simulink model "ABB_1010"  (R2024a)
settings: Solver=VariableStepAuto  StartTime=0.0  StopTime=200  RelTol=1e-3
model workspace: external: MATLAB File C:\Users\lucas\OneDrive\Documents\MATLAB\projeto final\ABB_1010_DataFile.m (data not in the file)
values from neighbouring files (symbols this model uses):
  g = 9.81    [inicializacaoAntropomorfico.m]
  I1 = [ 0.00243841  0.00000307  0.00007261    [inicializacaoAntropomorfico.m]
  I2 = [ 0.01633569  0.00000387 -0.00034405    [inicializacaoAntropomorfico.m]
  I3 = [ 0.00244760 -0.00000208  0.00000538    [inicializacaoAntropomorfico.m]
  I4 = [ 0.00245792 -0.00000008  0.00003121    [inicializacaoAntropomorfico.m]
  I5 = [ 0.00062165 -0.00000206 -0.00000303    [inicializacaoAntropomorfico.m]
  I6 = [ 0.00000357  0.00000000  0.00000000    [inicializacaoAntropomorfico.m]
  I7 = [(m7*L7^2)/12 0.00000000  0.00000000    [inicializacaoAntropomorfico.m]
  L = [L1, L2, L3, L4, L5, L6, L7]    [inicializacaoAntropomorfico.m]
  Lcm1 = [-0.00258308  0.00024508 -0.01434968]    [inicializacaoAntropomorfico.m]
  Lcm2 = [-0.02078894  0.00020016 -0.10516734]    [inicializacaoAntropomorfico.m]
  Lcm3 = [ 0.00021912  0.00015355 -0.06228290]    [inicializacaoAntropomorfico.m]
  Lcm4 = [-0.00172658 -0.00124140 -0.07369196]    [inicializacaoAntropomorfico.m]
  Lcm5 = [-0.00014110  0.00085992 -0.03825278]    [inicializacaoAntropomorfico.m]
  Lcm6 = [ 0.00002478  0.00000000 -0.00042157]    [inicializacaoAntropomorfico.m]
  Lcm7 = [ 0           0          -0.05000000]    [inicializacaoAntropomorfico.m]
  m = [m1, m2, m3, m4, m5, m6, m7]    [inicializacaoAntropomorfico.m]
  Pf = [  0.05    [inicializacaoAntropomorfico.m]
  Pi = [  0.2    [inicializacaoAntropomorfico.m]
  Raio = [0]    [inicializacaoAntropomorfico.m]
  Sentido = [0]    [inicializacaoAntropomorfico.m]
  Tipo = [1]    [inicializacaoAntropomorfico.m]
undefined symbols (not defined in the file or in its folder): smiData, X, Y, Z
libraries: sm_lib x35, nesl_utility x7
(part 6 of 16)

== matlab function ABB_1010/Dinamica/MATLAB Function1 ==
  data: H output; Q input; I1 parameter; I2 parameter; L parameter; Lcm1 parameter; Lcm2 parameter; Lcm3 parameter; Lcm4 parameter; Lcm5 parameter; Lcm6 parameter; I6 parameter; I5 parameter; I4 parameter; I3 parameter; dQ input; m parameter
function H = func_H(Q, I1, I2, L, Lcm1, Lcm2, Lcm3, Lcm4, Lcm5, Lcm6, I6, I5, I4, I3, dQ, m)
%func_H
%    OUT1 = func_H(Ixx2,Ixx3,Ixx4,Ixx5,Ixx6,Ixy2,Ixy3,Ixy4,Ixy5,Ixy6,Ixz2,Ixz3,Ixz4,Ixz5,Ixz6,Iyx2,Iyx3,Iyx4,Iyx5,Iyx6,Iyy4,Iyy5,Iyy6,Iyz2,Iyz3,Iyz4,Iyz5,Iyz6,Izx2,Izx3,Izx4,Izx5,Izx6,Izy2,Izy3,Izy4,Izy5,Izy6,Izz2,Izz3,Izz4,Izz5,Izz6,Lx2,Lx3,Lxcm2,Lxcm3,Lxcm4,Lxcm5,Lxcm6,Lycm2,Lycm3,Lycm4,Lycm5,Lycm6,Lz4,Lz5,Lzcm2,Lzcm3,Lzcm4,Lzcm5,Lzcm6,Q1,Q2,Q3,Q4,Q5,Q6,dQ1,dQ2,dQ3,dQ4,dQ5,dQ6,M2,M3,M4,M5,M6)

%    This function was generated by the Symbolic Math Toolbox version 24.1.
%    30-Apr-2025 06:22:27

m1  = m(1);
m2  = m(2);
m3  = m(3);
m4  = m(4);
m5  = m(5);
m6  = m(6);

Q1  = Q(1);
Q2  = Q(2);
Q3  = Q(3);
Q4  = Q(4);
Q5  = Q(5);
Q6  = Q(6);

dQ1 = dQ(1);
dQ2 = dQ(2);
dQ3 = dQ(3);
dQ4 = dQ(4);
dQ5 = dQ(5);
dQ6 = dQ(6);

Lz1 = L(1);
Lx2 = L(2);
Lx3 = L(3);
Lz4 = L(4);
Lz5 = L(5);
Lz6 = L(6);

Lxcm1 = Lcm1(1);
Lycm1 = Lcm1(2);
Lzcm1 = Lcm1(3);

Lxcm2 = Lcm2(1);
Lycm2 = Lcm2(2);
Lzcm2 = Lcm2(3);

Lxcm3 = Lcm3(1);
Lycm3 = Lcm3(2);
Lzcm3 = Lcm3(3);

Lxcm4 = Lcm4(1);
Lycm4 = Lcm4(2);
Lzcm4 = Lcm4(3);

Lxcm5 = Lcm5(1);
Lycm5 = Lcm5(2);
Lzcm5 = Lcm5(3);

Lxcm6 = Lcm6(1);
Lycm6 = Lcm6(2);
Lzcm6 = Lcm6(3);

Ixx1 = I1(1,1);
Ixy1 = I1(1,2);
Ixz1 = I1(1,3);
Iyx1 = I1(2,1);
Iyy1 = I1(2,2);
Iyz1 = I1(2,3);
Izx1 = I1(3,1);
Izy1 = I1(3,2);
Izz1 = I1(3,3);

Ixx2 = I2(1,1);
Ixy2 = I2(1,2);
Ixz2 = I2(1,3);
Iyx2 = I2(2,1);
Iyy2 = I2(2,2);
Iyz2 = I2(2,3);
Izx2 = I2(3,1);
Izy2 = I2(3,2);
Izz2 = I2(3,3);

Ixx3 = I3(1,1);
Ixy3 = I3(1,2);
Ixz3 = I3(1,3);
Iyx3 = I3(2,1);
Iyy3 = I3(2,2);
Iyz3 = I3(2,3);
Izx3 = I3(3,1);
Izy3 = I3(3,2);
Izz3 = I3(3,3);

Ixx4 = I4(1,1);
Ixy4 = I4(1,2);
Ixz4 = I4(1,3);
Iyx4 = I4(2,1);
Iyy4 = I4(2,2);
Iyz4 = I4(2,3);
Izx4 = I4(3,1);
Izy4 = I4(3,2);
Izz4 = I4(3,3);

Ixx5 = I5(1,1);
Ixy5 = I5(1,2);
Ixz5 = I5(1,3);
Iyx5 = I5(2,1);
Iyy5 = I5(2,2);
Iyz5 = I5(2,3);
Izx5 = I5(3,1);
Izy5 = I5(3,2);
Izz5 = I5(3,3);

Ixx6 = I6(1,1);
Ixy6 = I6(1,2);
Ixz6 = I6(1,3);
Iyx6 = I6(2,1);
Iyy6 = I6(2,2);
Iyz6 = I6(2,3);
Izx6 = I6(3,1);
Izy6 = I6(3,2);
Izz6 = I6(3,3);


t2 = cos(Q1);
t3 = cos(Q2);
t4 = cos(Q3);
t5 = cos(Q4);
t6 = cos(Q5);
t7 = cos(Q6);
t8 = sin(Q1);
t9 = sin(Q2);
t10 = sin(Q3);
t11 = sin(Q4);
t12 = sin(Q5);
t13 = sin(Q6);
t14 = Q2+Q3;
t15 = Lxcm4.^2;
t16 = Lxcm5.^2;
t17 = Lxcm6.^2;
t18 = Lycm4.^2;
t19 = Lycm5.^2;
t20 = Lycm6.^2;
t21 = Lz5.^2;
t22 = Lzcm5.^2;
t23 = Lzcm6.^2;
t24 = Q4.*2.0;
t25 = Q5.*2.0;
t26 = Q6.*2.0;
t27 = dQ1.^2;
t28 = dQ2.^2;
t29 = dQ3.^2;
t30 = dQ4.^2;
t31 = dQ5.^2;
t32 = dQ6.^2;
t33 = cos(t24);
t34 = cos(t25);
t35 = cos(t26);
t36 = t5.^2;
t37 = t6.^2;
t38 = t7.^2;
t39 = sin(t26);
t40 = t11.^2;
t41 = t12.^2;
t42 = t13.^2;
t43 = Lycm3.*t2;
t44 = Lzcm2.*t3;
t45 = cos(t14);
t46 = Lx2.*t9;
t47 = Lxcm2.*t9;
t48 = Lycm3.*t8;
t49 = sin(t14);
t50 = t2.*t5;
t51 = Lz4.*m5.*t4;
t52 = Lz4.*m6.*t4;
t53 = Lzcm3.*m3.*t4;
t54 = Lzcm4.*m4.*t4;
t55 = t2.*t11;
t56 = t5.*t8;
t57 = Lx3.*m4.*t10;
t58 = Lx3.*m5.*t10;
t59 = Lx3.*m6.*t10;
t60 = Lxcm3.*m3.*t10;
t61 = t8.*t11;
t72 = Lx2.*t2.*t3;
t75 = Lx3.*Lycm4.*m4.*t5;
t76 = Lx3.*Lycm5.*m5.*t5;
t77 = Lx3.*Lz5.*m6.*t6;
t78 = Lx3.*Lzcm5.*m5.*t6;
t79 = Lxcm5.*Lz4.*m5.*t6;
t80 = Lx3.*Lzcm6.*m6.*t6;
t81 = Lxcm4.*Lzcm4.*m4.*t5;
t82 = Lxcm5.*Lzcm5.*m5.*t5;
t92 = Ixx4.*t5.*t11;
t93 = Ixx6.*t5.*t11;
t94 = Ixx5.*t6.*t12;
t95 = Iyy4.*t5.*t11;
t96 = Iyy5.*t5.*t11;
t97 = Iyy6.*t6.*t12;
t98 = Izz5.*t5.*t11;
t99 = Izz6.*t5.*t11;
t100 = Izz5.*t6.*t12;
t101 = Izz6.*t6.*t12;
t102 = Lx2.*t3.*t8;
t103 = Lx3.*t3.*t10;
t104 = Lx3.*t4.*t9;
t108 = Lx3.*Lxcm4.*m4.*t11;
t109 = Lx3.*Lxcm5.*m5.*t12;
t110 = Lycm5.*Lz4.*m5.*t11;
t111 = Lycm4.*Lzcm4.*m4.*t11;
t112 = Lz4.*Lz5.*m6.*t12;
t113 = Lz4.*Lzcm5.*m5.*t12;
t114 = Lz4.*Lzcm6.*m6.*t12;
t119 = (Ixz4.*t5)./2.0;
t120 = (Ixz5.*t5)./2.0;
t121 = (Izx4.*t5)./2.0;
t122 = (Izx5.*t5)./2.0;
t123 = (Iyz4.*t11)./2.0;
t124 = (Izy4.*t11)./2.0;
t126 = t2.*t3.*t4;
t127 = Lz5.*m6.*t4.*t6;
t128 = Lzcm5.*m5.*t4.*t6;
t129 = Lzcm6.*m6.*t4.*t6;
t132 = t2.*t3.*t10;
t133 = t2.*t4.*t9;
t134 = t3.*t4.*t8;
t135 = Lxcm4.*m4.*t5.*t10;
t136 = Lxcm5.*m5.*t4.*t12;
t138 = t2.*t9.*t10;
t139 = t3.*t8.*t10;
t140 = t4.*t8.*t9;
t141 = Lycm4.*m4.*t10.*t11;
t142 = Lycm5.*m5.*t10.*t11;
t143 = t8.*t9.*t10;
t193 = Lx3.*Lycm6.*m6.*t5.*t7;
t198 = Lxcm6.*Lz4.*m6.*t6.*t7;
t199 = Lxcm6.*Lz5.*m6.*t5.*t7;
t200 = Lxcm6.*Lzcm6.*m6.*t5.*t7;
t230 = Lxcm4.*t3.*t5.*t10;
t231 = Lxcm4.*t4.*t5.*t9;
t236 = Lx3.*Lxcm5.*m5.*t6.*t11;
t237 = Lx3.*Lxcm6.*m6.*t5.*t13;
t238 = Lx3.*Lxcm6.*m6.*t7.*t11;
t239 = Lx3.*Lxcm6.*m6.*t7.*t12;
t240 = Lycm6.*Lz4.*m6.*t7.*t11;
t241 = Lycm6.*Lz4.*m6.*t6.*t13;
t242 = Lycm6.*Lz4.*m6.*t7.*t12;
t243 = Lycm6.*Lz5.*m6.*t5.*t13;
t244 = Lycm6.*Lz5.*m6.*t7.*t12;
t245 = Lycm5.*Lzcm5.*m5.*t6.*t11;
t246 = Lycm6.*Lzcm6.*m6.*t5.*t13;
t247 = Lycm6.*Lzcm6.*m6.*t7.*t12;
t266 = Lycm4.*t3.*t10.*t11;
t267 = Lycm4.*t4.*t9.*t11;
t268 = Lycm5.*t3.*t10.*t11;
t269 = Lycm5.*t4.*t9.*t11;
t273 = Lx3.*Lycm6.*m6.*t11.*t13;
t274 = Lx3.*Lycm6.*m6.*t12.*t13;
t275 = Lxcm5.*Lycm5.*m5.*t11.*t12;
t276 = Lxcm6.*Lycm6.*m6.*t11.*t12;
t277 = Lx3.*Lz5.*m6.*t11.*t12;
t278 = Lx3.*Lzcm5.*m5.*t11.*t12;
t279 = Lx3.*Lzcm6.*m6.*t11.*t12;
t280 = Lxcm6.*Lz4.*m6.*t11.*t13;
t281 = Lxcm6.*Lz4.*m6.*t12.*t13;
t282 = Lxcm6.*Lz5.*m6.*t12.*t13;
t283 = Lxcm6.*Lzcm6.*m6.*t12.*t13;
t288 = (Ixz6.*t5.*t7)./2.0;
t289 = (Izx6.*t5.*t7)./2.0;
t290 = (Iyz5.*t6.*t11)./2.0;
t291 = (Iyz6.*t5.*t13)./2.0;
t292 = (Iyz6.*t7.*t12)./2.0;
t293 = (Izy5.*t6.*t11)./2.0;
t294 = (Izy6.*t5.*t13)./2.0;
t295 = (Izy6.*t7.*t12)./2.0;
t297 = (Ixy5.*t11.*t12)./2.0;
t298 = (Ixy6.*t11.*t12)./2.0;
t299 = (Ixz6.*t12.*t13)./2.0;
t300 = (Iyx5.*t11.*t12)./2.0;
t301 = (Iyx6.*t11.*t12)./2.0;
t302 = (Izx6.*t12.*t13)./2.0;
t308 = Lxcm5.*m5.*t5.*t6.*t10;
t309 = Lxcm6.*m6.*t4.*t7.*t12;
t316 = Lycm6.*m6.*t7.*t10.*t11;
t317 = Lycm6.*m6.*t4.*t12.*t13;
t318 = Lz5.*m6.*t5.*t10.*t12;
t319 = Lzcm5.*m5.*t5.*t10.*t12;
t320 = Lzcm6.*m6.*t5.*t10.*t12;
t323 = Lxcm6.*m6.*t10.*t11.*t13;
t334 = Lz5.*Lzcm6.*m6.*t5.*t11.*2.0;
t335 = Lz5.*Lzcm6.*m6.*t6.*t12.*2.0;
t336 = m4.*t5.*t11.*t15;
t337 = m5.*t6.*t12.*t16;
t338 = m6.*t5.*t11.*t17;
t339 = m4.*t5.*t11.*t18;
t340 = m5.*t5.*t11.*t19;
t341 = m6.*t6.*t12.*t20;
t342 = m6.*t5.*t11.*t21;
t343 = m6.*t6.*t12.*t21;
t344 = m5.*t5.*t11.*t22;
t345 = m5.*t6.*t12.*t22;
t346 = m6.*t5.*t11.*t23;
t347 = m6.*t6.*t12.*t23;
t417 = Lxcm5.*t3.*t5.*t6.*t10;
t418 = Lxcm5.*t4.*t5.*t6.*t9;
t428 = Lycm6.*Lz5.*m6.*t6.*t7.*t11;
t431 = Lycm6.*Lzcm6.*m6.*t6.*t7.*t11;
t456 = Ixy6.*t5.*t7.*t11.*t13;
t457 = Ixy6.*t6.*t7.*t12.*t13;
t458 = Ixz5.*t5.*t6.*t11.*t12;
t459 = Iyx6.*t5.*t7.*t11.*t13;
t460 = Iyx6.*t6.*t7.*t12.*t13;
t461 = Izx5.*t5.*t6.*t11.*t12;
t467 = Lzcm5.*t3.*t5.*t10.*t12;
t468 = Lzcm5.*t4.*t5.*t9.*t12;
t478 = Lxcm6.*Lz5.*m6.*t6.*t11.*t13;
t480 = Lxcm6.*Lzcm6.*m6.*t6.*t11.*t13;
t489 = Ixx6.*t7.*t11.*t12.*t13;
t490 = Iyy6.*t7.*t11.*t12.*t13;
t538 = Lycm6.*m6.*t5.*t6.*t10.*t13;
t578 = (Iyz6.*t6.*t7.*t11)./2.0;
t581 = (Izy6.*t6.*t7.*t11)./2.0;
t586 = (Ixz6.*t6.*t11.*t13)./2.0;
t590 = (Izx6.*t6.*t11.*t13)./2.0;
t599 = Lxcm6.*m6.*t5.*t6.*t7.*t10;
t648 = Ixz6.*t5.*t6.*t7.*t11.*t12;
t650 = Izx6.*t5.*t6.*t7.*t11.*t12;
t667 = Iyz6.*t5.*t6.*t11.*t12.*t13;
t668 = Izy6.*t5.*t6.*t11.*t12.*t13;
t711 = Lz5.*Lzcm6.*m6.*t5.*t6.*t12.*-2.0;
t742 = Ixy5.*t5.*t11.*t12.*(-1.0./2.0);
t743 = Iyx5.*t5.*t11.*t12.*(-1.0./2.0);
t788 = Lxcm6.*Lycm6.*m6.*t5.*t7.*t11.*t13.*2.0;
t789 = Lxcm6.*Lycm6.*m6.*t6.*t7.*t12.*t13.*2.0;
t791 = m6.*t7.*t11.*t12.*t13.*t17;
t792 = m6.*t7.*t11.*t12.*t13.*t20;
t886 = Ixz6.*t5.*t7.*t11.*t12.*(-1.0./2.0);
t887 = Izx6.*t5.*t7.*t11.*t12.*(-1.0./2.0);
t928 = Lxcm6.*Lycm6.*m6.*t5.*t6.*t7.*t11.*t13.*4.0;
t968 = Lxcm6.*Lycm6.*m6.*t5.*t6.*t7.*t12.*t13.*-2.0;
t62 = Ixx3.*t45;
t63 = Ixz3.*t45;
t64 = Izx3.*t45;
t65 = Izx4.*t45;
t66 = Izy4.*t45;
t67 = Izz3.*t45;
t68 = Izz4.*t45;
t69 = Lz4.*t45;
t70 = Lzcm3.*t45;
t71 = Lzcm4.*t45;
t73 = Lycm4.*t50;
t74 = Lycm5.*t50;
t83 = Ixx3.*t49;
t84 = Ixz3.*t49;
t85 = Izx3.*t49;
t86 = Izx4.*t49;
t87 = Izy4.*t49;
t88 = Izz3.*t49;
t89 = Izz4.*t49;
t90 = Lx3.*t49;
t91 = Lxcm3.*t49;
t105 = Lxcm4.*t55;
t106 = Lycm4.*t56;
t107 = Lycm5.*t56;
t115 = Lxcm4.*t61;
t116 = -t46;
t117 = -t47;
t118 = -t48;
t125 = t6.*t45;
t130 = t12.*t45;
t131 = t6.*t49;
t137 = t12.*t49;
t144 = -t50;
t145 = -t57;
t146 = -t58;
t147 = -t59;
t148 = -t60;
t149 = -t61;
t154 = -t77;
t155 = -t78;
t156 = -t80;
t157 = -t81;
t163 = -t92;
t164 = -t98;
t165 = -t99;
t166 = -t100;
t167 = -t101;
t171 = -t119;
t172 = -t121;
t173 = Ixz5.*t5.*t37;
t174 = Izx5.*t5.*t37;
t175 = Lxcm4.*Lycm4.*m4.*t33;
t176 = Lxcm6.*Lycm6.*m6.*t35;
t177 = Lxcm5.*Lzcm5.*m5.*t34;
t178 = Ixx4.*t5.*t45;
t179 = Ixy4.*t5.*t45;
t180 = Ixz4.*t5.*t45;
t186 = Lx3.*t2.*t45;
t187 = Lxcm3.*t2.*t45;
t191 = Lx3.*t126;
t192 = Lycm6.*t7.*t50;
t196 = t5.*t79;
t201 = Ixx4.*t5.*t49;
t203 = Ixy4.*t5.*t49;
t205 = Ixz4.*t5.*t49;
t207 = Iyx4.*t11.*t45;
t208 = Iyx5.*t11.*t45;
t209 = Iyy4.*t11.*t45;
t210 = Iyy5.*t11.*t45;
t211 = Iyz4.*t11.*t45;
t212 = Iyz5.*t11.*t45;
t219 = Lx3.*t8.*t45;
t220 = Lxcm3.*t8.*t45;
t222 = Lz4.*t2.*t49;
t223 = Lzcm3.*t2.*t49;
t224 = Lzcm4.*t2.*t49;
t225 = t5.*t94;
t226 = t5.*t97;
t227 = t5.*t100;
t228 = t5.*t101;
t229 = Lx3.*t134;
t232 = Lxcm5.*t6.*t55;
t233 = Lxcm6.*t13.*t50;
t234 = Lycm6.*t7.*t56;
t235 = t5.*t109;
t248 = t5.*t112;
t249 = t5.*t113;
t250 = t5.*t114;
t254 = Iyx4.*t11.*t49;
t255 = Iyx5.*t11.*t49;
t256 = Iyy4.*t11.*t49;
t257 = Iyy5.*t11.*t49;
t258 = Iyz4.*t11.*t49;
t259 = Iyz5.*t11.*t49;
t260 = Lz4.*t8.*t49;
t261 = Lzcm3.*t8.*t49;
t262 = Lzcm4.*t8.*t49;
t263 = Lx3.*t138;
t264 = Lxcm5.*t6.*t61;
t265 = Lxcm6.*t13.*t56;
t270 = Lz5.*t12.*t55;
t271 = Lzcm5.*t12.*t55;
t272 = Lzcm6.*t12.*t55;
t284 = Lx3.*t143;
t286 = Lzcm5.*t12.*t61;
t305 = t7.*t11.*t45;
t306 = t5.*t7.*t49;
t311 = t11.*t13.*t45;
t312 = t5.*t13.*t49;
t313 = t7.*t11.*t49;
t321 = t11.*t13.*t49;
t324 = -t135;
t325 = -t136;
t326 = -t138;
t327 = -t143;
t328 = (Ixy4.*t33)./2.0;
t329 = (Ixy6.*t35)./2.0;
t330 = (Ixz5.*t34)./2.0;
t331 = (Iyx4.*t33)./2.0;
t332 = (Iyx6.*t35)./2.0;
t333 = (Izx5.*t34)./2.0;
t348 = -t288;
t349 = -t289;
t350 = -t291;
t351 = -t294;
t352 = Ixz6.*t5.*t7.*t37;
t353 = Izx6.*t5.*t7.*t37;
t354 = Lxcm5.*Lycm5.*m5.*t6.*t36;
t355 = Lxcm6.*Lycm6.*m6.*t6.*t36;
t356 = Lxcm6.*Lz5.*m6.*t7.*t37;
t357 = Lxcm6.*Lzcm6.*m6.*t7.*t37;
t358 = -t297;
t359 = -t300;
t360 = Ixx5.*t5.*t11.*t37;
t361 = t36.*t94;
t362 = t38.*t93;
t363 = Ixx6.*t6.*t12.*t38;
t364 = Ixx6.*t7.*t13.*t36;
t365 = Ixx6.*t7.*t13.*t37;
t366 = Iyy6.*t5.*t11.*t37;
t367 = Iyy6.*t5.*t11.*t38;
t368 = t36.*t97;
t369 = t38.*t97;
t370 = Iyy6.*t7.*t13.*t36;
t371 = Iyy6.*t7.*t13.*t37;
t372 = Iyz6.*t5.*t13.*t37;
t373 = Izy6.*t5.*t13.*t37;
t374 = t37.*t98;
t375 = t36.*t100;
t376 = t37.*t99;
t377 = t36.*t101;
t378 = Lxcm5.*Lycm5.*m5.*t6.*t40;
t379 = Lxcm6.*Lycm6.*m6.*t6.*t40;
t380 = Lxcm6.*Lz5.*m6.*t7.*t41;
t381 = Lxcm6.*Lzcm6.*m6.*t7.*t41;
t382 = Lycm6.*Lz5.*m6.*t13.*t37;
t383 = Lycm5.*Lzcm5.*m5.*t12.*t36;
t384 = Lycm6.*Lzcm6.*m6.*t13.*t37;
t385 = Ixy6.*t11.*t12.*t38;
t386 = Iyx6.*t11.*t12.*t38;
t387 = Lycm6.*Lz5.*m6.*t13.*t41;
t388 = Lycm5.*Lzcm5.*m5.*t12.*t40;
t389 = Lycm6.*Lzcm6.*m6.*t13.*t41;
t395 = Lxcm4.*t3.*t4.*t50;
t396 = t6.*t193;
t397 = t5.*t198;
t416 = Lxcm4.*t3.*t4.*t56;
t419 = Lxcm6.*t6.*t7.*t55;
t420 = Lycm4.*t3.*t4.*t55;
t421 = Lycm5.*t3.*t4.*t55;
t422 = Lx2.*t308;
t423 = Lx2.*t309;
t424 = t6.*t237;
t425 = t5.*t239;
t426 = t6.*t238;
t427 = t5.*t241;
t429 = t6.*t244;
t430 = t5.*t245;
t432 = t6.*t247;
t466 = Lycm6.*t6.*t13.*t55;
t469 = Lx2.*t316;
t470 = Lx2.*t317;
t471 = t5.*t274;
t472 = t6.*t273;
t473 = t5.*t275;
t474 = t5.*t276;
t475 = Lx2.*t318;
t476 = Lx2.*t319;
t477 = Lx2.*t320;
t479 = t6.*t282;
t481 = t6.*t283;
t491 = Lxcm4.*t9.*t10.*t56;
t492 = Lycm4.*t9.*t10.*t55;
t493 = Lycm5.*t9.*t10.*t55;
t494 = Lycm6.*t6.*t13.*t61;
t495 = Lx2.*t323;
t496 = Lycm4.*t9.*t10.*t61;
t497 = Lycm5.*t9.*t10.*t61;
t506 = -t199;
t507 = -t200;
t512 = -t238;
t513 = -t239;
t514 = -t241;
t515 = -t243;
t516 = -t246;
t526 = -t266;
t527 = -t267;
t528 = -t268;
t529 = -t269;
t530 = -t274;
t531 = -t275;
t541 = t37.*t82.*2.0;
t543 = -t308;
t544 = -t309;
t546 = -t318;
t547 = -t319;
t548 = -t320;
t551 = (Ixy5.*t6.*t36)./2.0;
t552 = (Ixy6.*t6.*t36)./2.0;
t553 = (Ixz6.*t7.*t37)./2.0;
t554 = (Iyx5.*t6.*t36)./2.0;
t555 = (Iyx6.*t6.*t36)./2.0;
t556 = (Izx6.*t7.*t37)./2.0;
t557 = (Ixy5.*t6.*t40)./2.0;
t558 = (Ixy6.*t6.*t40)./2.0;
t559 = (Ixz6.*t7.*t41)./2.0;
t560 = (Iyx5.*t6.*t40)./2.0;
t561 = (Iyx6.*t6.*t40)./2.0;
t562 = (Iyz5.*t12.*t36)./2.0;
t563 = (Iyz6.*t13.*t37)./2.0;
t564 = (Izx6.*t7.*t41)./2.0;
t565 = (Izy5.*t12.*t36)./2.0;
t566 = (Izy6.*t13.*t37)./2.0;
t567 = (Iyz5.*t12.*t40)./2.0;
t568 = (Iyz6.*t13.*t41)./2.0;
t569 = (Izy5.*t12.*t40)./2.0;
t570 = (Izy6.*t13.*t41)./2.0;
t572 = t5.*t337;
t573 = t5.*t341;
t574 = t5.*t343;
t575 = t5.*t345;
t576 = t5.*t347;
t577 = t5.*t290;
t579 = t6.*t292;
t580 = t5.*t293;
t582 = t6.*t295;
t585 = t5.*t298;
t587 = t6.*t299;
t589 = t5.*t301;
t591 = t6.*t302;
t592 = -t337;
t593 = -t338;
t594 = -t339;
t595 = -t340;
t596 = -t341;
t600 = t36.*t282;
t601 = t36.*t283;
t602 = t40.*t244;
t603 = t40.*t247;
t604 = t40.*t282;
t605 = t40.*t283;
t613 = Lxcm5.*t3.*t4.*t6.*t50;
t633 = Lxcm5.*t3.*t4.*t6.*t56;
t634 = Lycm6.*t3.*t4.*t7.*t55;
t635 = Lz5.*t3.*t4.*t12.*t50;
t636 = Lzcm5.*t3.*t4.*t12.*t50;
t637 = Lzcm6.*t3.*t4.*t12.*t50;
t640 = Lx2.*t599;
t641 = t5.*t428;
t642 = t5.*t431;
t647 = t5.*t457;
t649 = t5.*t460;
t652 = Lxcm6.*t3.*t4.*t13.*t55;
t653 = Lxcm6.*t7.*t12.*t132;
t654 = Lxcm6.*t7.*t12.*t133;
t656 = Lz5.*t3.*t4.*t12.*t56;
t657 = Lzcm5.*t3.*t4.*t12.*t56;
t658 = Lzcm6.*t3.*t4.*t12.*t56;
t659 = Lx2.*t538;
t660 = t5.*t478;
t661 = t11.*t12.*t199;
t662 = t5.*t480;
t663 = t11.*t12.*t200;
t665 = t7.*t12.*t13.*t93;
H = ft_1({Ixx2,Ixx4,Ixx5,Ixx6,Ixy2,Ixy3,Ixy4,Ixy5,Ixy6,Ixz2,Ixz4,Ixz5,Ixz6,Iyx2,Iyx3,Iyx4,Iyx5,Iyx6,Iyy4,Iyy5,Iyy6,Iyz2,Iyz3,Iyz4,Iyz5,Iyz6,Izx2,Izx4,Izx5,Izx6,Izy2,Izy3,Izy4,Izy5,Izy6,Izz2,Izz5,Izz6,Lx2,Lx3,Lxcm2,Lxcm3,Lxcm4,Lxcm5,Lxcm6,Lycm2,Lycm3,Lycm4,Lycm5,Lycm6,Lz4,Lz5,Lzcm2,Lzcm3,Lzcm4,Lzcm5,Lzcm6,m2,m3,m4,m5,m6,t10,t100,t101,t102,t103,t104,t105,t106,t107,t108,t109,t11,t110,t111,t112,t113,t114,t115,t116,t117,t118,t12,t120,t122,t123,t124,t125,t126,t127,t128,t129,t13,t130,t131,t132,t133,t134,t136,t137,t139,t140,t141,t142,t144,t145,t146,t147,t148,t149,t154,t155,t156,t157,t16,t163,t164,t165,t166,t167,t17,t171,t172,t173,t174,t175,t176,t177,t178,t179,t180,t186,t187,t191,t192,t193,t196,t198,t199,t2,t20,t200,t201,t203,t205,t207,t208,t209,t210,t211,t212,t219,t220,t222,t223,t224,t225,t226,t227,t228,t229,t230,t231,t232,t233,t234,t235,t236,t237,t239,t240,t241,t242,t243,t244,t245,t246,t247,t248,t249,t250,t254,t255,t256,t257,t258,t259,t260,t261,t262,t263,t264,t265,t27,t270,t271,t272,t273,t274,t276,t277,t278,t279,t28,t280,t281,t282,t283,t284,t286,t288,t289,t29,t290,t291,t292,t293,t294,t295,t298,t299,t3,t30,t301,t302,t305,t306,t31,t311,t312,t313,t316,t317,t32,t321,t323,t324,t325,t326,t327,t328,t329,t330,t331,t332,t333,t334,t335,t336,t337,t338,t339,t340,t341,t342,t343,t344,t345,t346,t347,t348,t349,t350,t351,t352,t353,t354,t355,t356,t357,t358,t359,t36,t360,t361,t362,t363,t364,t365,t366,t367,t368,t369,t37,t370,t371,t372,t373,t374,t375,t376,t377,t378,t379,t38,t380,t381,t382,t383,t384,t385,t386,t387,t388,t389,t39,t395,t396,t397,t4,t40,t41,t416,t417,t418,t419,t42,t420,t421,t422,t423,t424,t425,t426,t427,t428,t429,t43,t430,t431,t432,t44,t45,t456,t457,t458,t459,t46,t460,t461,t466,t467,t468,t469,t470,t471,t472,t473,t474,t475,t476,t477,t478,t479,t480,t481,t489,t49,t490,t491,t492,t493,t494,t495,t496,t497,t5,t50,t506,t507,t51,t512,t513,t514,t515,t516,t52,t526,t527,t528,t529,t53,t530,t531,t538,t54,t541,t543,t544,t546,t547,t548,t55,t551,t552,t553,t554,t555,t556,t557,t558,t559,t56,t560,t561,t562,t563,t564,t565,t566,t567,t568,t569,t57,t570,t572,t573,t574,t575,t576,t577,t578,t579,t58,t580,t581,t582,t585,t586,t587,t589,t59,t590,t591,t592,t593,t594,t595,t596,t599,t6,t600,t601,t602,t603,t604,t605,t61,t613,t62,t63,t633,t634,t635,t636,t637,t64,t640,t641,t642,t647,t648,t649,t65,t650,t652,t653,t654,t656,t657,t658,t659,t66,t660,t661,t662,t663,t665,t667,t668,t67,t68,t69,t7,t70,t71,t711,t72,t73,t74,t742,t743,t75,t76,t788,t789,t79,t791,t792,t8,t82,t83,t84,t85,t86,t87,t88,t886,t887,t89,t9,t90,t91,t92,t928,t93,t94,t95,t96,t968,t97,t98,t99});
end
function out1 = ft_1(ct)
[Ixx2,Ixx4,Ixx5,Ixx6,Ixy2,Ixy3,Ixy4,Ixy5,Ixy6,Ixz2,Ixz4,Ixz5,Ixz6,Iyx2,Iyx3,Iyx4,Iyx5,Iyx6,Iyy4,Iyy5,Iyy6,Iyz2,Iyz3,Iyz4,Iyz5,Iyz6,Izx2,Izx4,Izx5,Izx6,Izy2,Izy3,Izy4,Izy5,Izy6,Izz2,Izz5,Izz6,Lx2,Lx3,Lxcm2,Lxcm3,Lxcm4,Lxcm5,Lxcm6,Lycm2,Lycm3,Lycm4,Lycm5,Lycm6,Lz4,Lz5,Lzcm2,Lzcm3,Lzcm4,Lzcm5,Lzcm6,m2,m3,m4,m5,m6,t10,t100,t101,t102,t103,t104,t105,t106,t107,t108,t109,t11,t110,t111,t112,t113,t114,t115,t116,t117,t118,t12,t120,t122,t123,t124,t125,t126,t127,t128,t129,t13,t130,t131,t132,t133,t134,t136,t137,t139,t140,t141,t142,t144,t145,t146,t147,t148,t149,t154,t155,t156,t157,t16,t163,t164,t165,t166,t167,t17,t171,t172,t173,t174,t175,t176,t177,t178,t179,t180,t186,t187,t191,t192,t193,t196,t198,t199,t2,t20,t200,t201,t203,t205,t207,t208,t209,t210,t211,t212,t219,t220,t222,t223,t224,t225,t226,t227,t228,t229,t230,t231,t232,t233,t234,t235,t236,t237,t239,t240,t241,t242,t243,t244,t245,t246,t247,t248,t249,t250,t254,t255,t256,t257,t258,t259,t260,t261,t262,t263,t264,t265,t27,t270,t271,t272,t273,t274,t276,t277,t278,t279,t28,t280,t281,t282,t283,t284,t286,t288,t289,t29,t290,t291,t292,t293,t294,t295,t298,t299,t3,t30,t301,t302,t305,t306,t31,t311,t312,t313,t316,t317,t32,t321,t323,t324,t325,t326,t327,t328,t329,t330,t331,t332,t333,t334,t335,t336,t337,t338,t339,t340,t341,t342,t343,t344,t345,t346,t347,t348,t349,t350,t351,t352,t353,t354,t355,t356,t357,t358,t359,t36,t360,t361,t362,t363,t364,t365,t366,t367,t368,t369,t37,t370,t371,t372,t373,t374,t375,t376,t377,t378,t379,t38,t380,t381,t382,t383,t384,t385,t386,t387,t388,t389,t39,t395,t396,t397,t4,t40,t41,t416,t417,t418,t419,t42,t420,t421,t422,t423,t424,t425,t426,t427,t428,t429,t43,t430,t431,t432,t44,t45,t456,t457,t458,t459,t46,t460,t461,t466,t467,t468,t469,t470,t471,t472,t473,t474,t475,t476,t477,t478,t479,t480,t481,t489,t49,t490,t491,t492,t493,t494,t495,t496,t497,t5,t50,t506,t507,t51,t512,t513,t514,t515,t516,t52,t526,t527,t528,t529,t53,t530,t531,t538,t54,t541,t543,t544,t546,t547,t548,t55,t551,t552,t553,t554,t555,t556,t557,t558,t559,t56,t560,t561,t562,t563,t564,t565,t566,t567,t568,t569,t57,t570,t572,t573,t574,t575,t576,t577,t578,t579,t58,t580,t581,t582,t585,t586,t587,t589,t59,t590,t591,t592,t593,t594,t595,t596,t599,t6,t600,t601,t602,t603,t604,t605,t61,t613,t62,t63,t633,t634,t635,t636,t637,t64,t640,t641,t642,t647,t648,t649,t65,t650,t652,t653,t654,t656,t657,t658,t659,t66,t660,t661,t662,t663,t665,t667,t668,t67,t68,t69,t7,t70,t71,t711,t72,t73,t74,t742,t743,t75,t76,t788,t789,t79,t791,t792,t8,t82,t83,t84,t85,t86,t87,t88,t886,t887,t89,t9,t90,t91,t92,t928,t93,t94,t95,t96,t968,t97,t98,t99] = ct{:};
t666 = t5.*t490;
t669 = Lxcm5.*t6.*t9.*t10.*t56;
t671 = Lycm6.*t7.*t9.*t10.*t55;
t672 = Lycm6.*t12.*t13.*t132;
t673 = Lycm6.*t12.*t13.*t133;
t677 = t11.*t12.*t243;
t678 = t11.*t12.*t246;
t682 = Lxcm6.*t9.*t10.*t13.*t55;
t683 = Lycm6.*t7.*t9.*t10.*t61;
t684 = Lz5.*t9.*t10.*t12.*t56;
t685 = Lzcm5.*t9.*t10.*t12.*t56;
t686 = Lzcm6.*t9.*t10.*t12.*t56;
t695 = Lxcm6.*t9.*t10.*t13.*t61;
t698 = Ixy6.*t6.*t36.*t38;
t699 = Iyx6.*t6.*t36.*t38;
t702 = Lxcm6.*Lycm6.*m6.*t36.*t38;
t703 = Lxcm6.*Lycm6.*m6.*t37.*t38;
t704 = Lxcm5.*Lzcm5.*m5.*t36.*t37;
t712 = Ixy6.*t6.*t38.*t40;
t713 = Iyx6.*t6.*t38.*t40;
t722 = -t456;
t723 = -t459;
t724 = Lxcm6.*Lycm6.*m6.*t36.*t42;
t725 = Lxcm6.*Lycm6.*m6.*t37.*t42;
t726 = Lxcm5.*Lzcm5.*m5.*t36.*t41;
t740 = -t490;
t750 = t36.*t244;
t751 = t36.*t247;
t752 = t6.*t42.*t93;
t753 = Ixx6.*t6.*t7.*t13.*t40;
t756 = Iyy6.*t5.*t6.*t11.*t42;
t757 = Iyy6.*t6.*t7.*t13.*t40;
t758 = t38.*t276.*2.0;
t759 = m5.*t5.*t11.*t16.*t37;
t760 = t36.*t337;
t761 = t38.*t338;
t762 = m6.*t6.*t12.*t17.*t38;
t763 = m6.*t7.*t13.*t17.*t36;
t764 = m6.*t7.*t13.*t17.*t37;
t765 = m6.*t5.*t11.*t20.*t37;
t766 = m6.*t5.*t11.*t20.*t38;
t767 = t36.*t341;
t768 = t38.*t341;
t769 = m6.*t7.*t13.*t20.*t36;
t770 = m6.*t7.*t13.*t20.*t37;
t771 = t37.*t342;
t772 = t36.*t343;
t773 = t37.*t344;
t774 = t36.*t345;
t775 = t37.*t346;
t776 = t36.*t347;
t778 = t36.*t292;
t779 = t36.*t295;
t780 = t36.*t299;
t782 = t36.*t302;
t784 = t6.*t456.*2.0;
t785 = t6.*t459.*2.0;
t790 = t6.*t11.*t12.*t82.*2.0;
t793 = t5.*t578;
t794 = t5.*t581;
t797 = t5.*t586;
t799 = t5.*t590;
t804 = t11.*t12.*t291;
t805 = t11.*t12.*t294;
t806 = (Ixy6.*t36.*t38)./2.0;
t807 = (Ixy6.*t37.*t38)./2.0;
t808 = (Ixz5.*t36.*t37)./2.0;
t809 = (Iyx6.*t36.*t38)./2.0;
t810 = (Iyx6.*t37.*t38)./2.0;
t811 = (Izx5.*t36.*t37)./2.0;
t812 = (Ixy6.*t36.*t42)./2.0;
t813 = (Ixy6.*t37.*t42)./2.0;
t814 = (Ixz5.*t36.*t41)./2.0;
t815 = (Iyx6.*t36.*t42)./2.0;
t816 = (Iyx6.*t37.*t42)./2.0;
t817 = (Izx5.*t36.*t41)./2.0;
t819 = t37.*t199.*2.0;
t820 = t37.*t200.*2.0;
t821 = t37.*t243.*2.0;
t822 = t37.*t246.*2.0;
t823 = t37.*t334;
t825 = -t599;
t830 = Lycm6.*t3.*t4.*t6.*t13.*t56;
t833 = Lxcm6.*t6.*t7.*t9.*t10.*t56;
t834 = Lycm6.*t6.*t9.*t10.*t13.*t50;
t835 = Lycm6.*t6.*t9.*t10.*t13.*t56;
t843 = Iyz6.*t7.*t12.*t40.*(-1.0./2.0);
t844 = Izy6.*t7.*t12.*t40.*(-1.0./2.0);
t863 = Ixz6.*t12.*t13.*t40.*(-1.0./2.0);
t864 = Izx6.*t12.*t13.*t40.*(-1.0./2.0);
t865 = -t788;
t870 = -t667;
t871 = -t668;
t891 = t37.*t456;
t892 = t36.*t457;
t893 = t37.*t459;
t894 = t36.*t460;
t905 = Lxcm6.*t3.*t4.*t6.*t7.*t50;
t909 = Lz5.*Lzcm6.*m6.*t5.*t11.*t37.*-2.0;
t910 = Lz5.*Lzcm6.*m6.*t6.*t12.*t36.*-2.0;
t911 = Lxcm6.*t3.*t4.*t6.*t7.*t56;
t934 = t5.*t792;
t937 = t132+t133;
t938 = -t791;
t948 = t139+t140;
t958 = t6.*t42.*t338;
t959 = m6.*t6.*t7.*t13.*t17.*t40;
t960 = m6.*t5.*t6.*t11.*t20.*t42;
t961 = m6.*t6.*t7.*t13.*t20.*t40;
t980 = Ixz6.*t7.*t36.*t37.*(-1.0./2.0);
t981 = Izx6.*t7.*t36.*t37.*(-1.0./2.0);
t983 = Iyz6.*t13.*t36.*t41.*(-1.0./2.0);
t984 = Izy6.*t13.*t36.*t41.*(-1.0./2.0);
t995 = Iyz6.*t6.*t7.*t12.*t36.*(-1.0./2.0);
t996 = Izy6.*t6.*t7.*t12.*t36.*(-1.0./2.0);
t998 = Ixz6.*t6.*t12.*t13.*t36.*(-1.0./2.0);
t999 = Izx6.*t6.*t12.*t13.*t36.*(-1.0./2.0);
t1024 = Lxcm6.*Lycm6.*m6.*t5.*t7.*t11.*t13.*t37.*-2.0;
t1031 = Ixy6.*t36.*t37.*t38.*(-1.0./2.0);
t1032 = Iyx6.*t36.*t37.*t38.*(-1.0./2.0);
t150 = -t66;
t151 = -t69;
t152 = -t70;
t153 = -t71;
t158 = -t85;
t159 = -t86;
t160 = -t88;
t161 = -t90;
t162 = -t91;
t168 = -t106;
t169 = -t107;
t170 = -t115;
t181 = Izx5.*t125;
t182 = Izx6.*t125;
t183 = Izy5.*t125;
t184 = Izy6.*t125;
t185 = Izz5.*t125;
t188 = Lz5.*t125;
t189 = Lzcm5.*t125;
t190 = Lzcm6.*t125;
t202 = Ixx5.*t130;
t204 = Ixy5.*t130;
t206 = Ixz5.*t130;
t213 = Izx5.*t131;
t214 = Izx6.*t131;
t215 = Izy5.*t131;
t216 = Izy6.*t131;
t217 = Izz5.*t131;
t218 = Izz6.*t131;
t221 = Lxcm5.*t130;
t251 = Ixx5.*t137;
t252 = Ixy5.*t137;
t253 = Ixz5.*t137;
t296 = t5.*t125;
t303 = t5.*t130;
t304 = t5.*t131;
t307 = t7.*t130;
t310 = t5.*t137;
t314 = t13.*t130;
t315 = t7.*t137;
t322 = t13.*t137;
t390 = -t173;
t391 = -t174;
t403 = Iyx6.*t305;
t404 = Iyy6.*t305;
t405 = Iyz6.*t305;
t413 = Lz5.*t2.*t131;
t414 = Lzcm5.*t2.*t131;
t415 = Lzcm6.*t2.*t131;
t433 = Ixx6.*t311;
t435 = Ixy6.*t311;
t437 = Ixz6.*t311;
t439 = Iyx6.*t313;
t441 = Iyy6.*t313;
t448 = Lxcm5.*t2.*t137;
t449 = Lycm6.*t313;
t451 = Lz5.*t8.*t131;
t453 = Lzcm5.*t8.*t131;
t454 = Lzcm6.*t8.*t131;
t482 = Ixx6.*t321;
t483 = Ixy6.*t321;
t487 = Lxcm5.*t8.*t137;
t488 = Lxcm6.*t321;
t498 = -t180;
t502 = t5.*t154;
t503 = t5.*t155;
t504 = -t196;
t505 = t5.*t156;
t508 = -t208;
t509 = -t225;
t510 = -t226;
t511 = -t234;
t517 = -t248;
t518 = -t249;
t519 = -t250;
t521 = -t258;
t522 = -t259;
t523 = -t263;
t524 = Lxcm5.*t6.*t149;
t525 = -t265;
t532 = -t284;
t533 = Lz5.*t12.*t149;
t534 = Lzcm5.*t12.*t149;
t535 = Lzcm6.*t12.*t149;
t537 = t7.*t11.*t131;
t539 = t11.*t13.*t131;
t542 = t44+t117;
t549 = -t321;
t606 = -t352;
t607 = -t353;
t611 = -t355;
t612 = -t541;
t614 = -t360;
t615 = -t361;
t616 = -t362;
t617 = -t365;
t618 = -t366;
t619 = -t368;
t620 = -t369;
t621 = -t370;
t627 = -t378;
t628 = -t380;
t629 = -t381;
t630 = -t382;
t631 = -t384;
t638 = -t385;
t639 = -t386;
t645 = -t388;
t680 = -t552;
t681 = -t555;
t689 = -t557;
t690 = -t559;
t691 = -t560;
t692 = -t563;
t693 = -t564;
t694 = -t566;
t696 = -t396;
t697 = -t397;
t705 = -t420;
t706 = -t421;
t707 = -t567;
t708 = -t569;
t709 = -t424;
t710 = -t427;
t727 = Lxcm4.*t9.*t10.*t144;
t728 = Lxcm6.*t6.*t7.*t149;
t729 = Lycm4.*t3.*t4.*t149;
t730 = Lycm5.*t3.*t4.*t149;
t731 = -t466;
t732 = -t471;
t733 = -t472;
t734 = -t473;
t741 = -t491;
t744 = t6.*t362;
t745 = t5.*t363;
t746 = t6.*t364;
t747 = t6.*t367;
t748 = t38.*t226;
t749 = t6.*t370;
t795 = t64+t83;
t796 = t67+t84;
t801 = -t574;
t802 = -t575;
t803 = -t576;
t826 = -t758;
t827 = -t602;
t828 = -t603;
t831 = -t604;
t832 = -t605;
t840 = t36.*t356;
t841 = t36.*t357;
t842 = -t634;
t845 = -t640;
t846 = t37.*t362;
t847 = t36.*t363;
t848 = t37.*t364;
t849 = t38.*t366;
t850 = t38.*t368;
t852 = -t647;
t853 = -t649;
t854 = t36.*t380;
t855 = t36.*t381;
t856 = t36.*t382;
t857 = t36.*t384;
t858 = Lxcm5.*t6.*t9.*t10.*t144;
t859 = -t652;
t860 = -t653;
t861 = -t654;
t862 = Lycm6.*t3.*t4.*t7.*t149;
t866 = t11.*t12.*t506;
t867 = t11.*t12.*t507;
t869 = -t666;
t872 = t36.*t387;
t873 = t36.*t389;
t874 = -t669;
t875 = Lxcm6.*t3.*t4.*t13.*t149;
t876 = Lz5.*t9.*t10.*t12.*t144;
t877 = Lzcm5.*t9.*t10.*t12.*t144;
t878 = Lzcm6.*t9.*t10.*t12.*t144;
t879 = -t684;
t880 = -t685;
t881 = -t686;
t882 = -t702;
t883 = -t704;
t884 = -t712;
t885 = -t713;
t888 = -t725;
t889 = t36.*t429;
t890 = t36.*t432;
t895 = t36.*t479;
t896 = t36.*t481;
t897 = -t806;
t898 = -t808;
t899 = -t809;
t900 = -t811;
t901 = -t813;
t902 = -t816;
t903 = -t819;
t904 = -t820;
t913 = -t752;
t916 = -t757;
t917 = -t762;
t918 = -t763;
t919 = -t766;
t920 = -t770;
t921 = -t771;
t922 = -t772;
t923 = -t773;
t924 = -t774;
t925 = -t775;
t926 = -t776;
t929 = t6.*t661.*2.0;
t930 = t6.*t663.*2.0;
t931 = t6.*t677.*2.0;
t932 = t6.*t678.*2.0;
t935 = t38.*t355.*2.0;
t936 = t38.*t379.*2.0;
t944 = t36.*t559;
t945 = t36.*t563;
t946 = t36.*t564;
t947 = t36.*t566;
t951 = t38.*t474.*2.0;
t953 = t5.*t762;
t954 = t6.*t763;
t955 = t6.*t766;
t956 = t38.*t573;
t957 = t6.*t769;
t966 = Lxcm6.*t6.*t7.*t9.*t10.*t144;
t967 = -t830;
t969 = -t833;
t987 = t37.*t722;
t988 = -t892;
t989 = t37.*t723;
t990 = -t894;
t991 = t37.*t724;
t997 = Lycm6.*t3.*t4.*t6.*t13.*t144;
t1000 = t37.*t761;
t1001 = t36.*t762;
t1003 = t38.*t765;
t1005 = t37.*t769;
t1006 = Lz4.*t937;
t1009 = t7.*t12.*t13.*t593;
t1010 = Lz4.*t948;
t1012 = t7.*t12.*t13.*t355.*2.0;
t1013 = t126+t326;
t1014 = t134+t327;
t1015 = t6.*t38.*t593;
t1018 = -t959;
t1019 = -t960;
t1022 = t37.*t812;
t1023 = t37.*t815;
t1026 = t6.*t937;
t1027 = t12.*t937;
t1029 = t6.*t948;
t1030 = t12.*t948;
t1036 = t36.*t38.*t596;
t1058 = t87+t179+t209;
t1059 = t65+t201+t254;
t1070 = t43+t102+t220+t261;
t1074 = t72+t118+t187+t223;
t1179 = t51+t52+t53+t54+t127+t128+t129+t141+t142+t145+t146+t147+t148+t316+t317+t323+t324+t325+t538+t543+t544+t546+t547+t548+t825;
t392 = Ixx5.*t296;
t393 = Ixy5.*t296;
t394 = Ixz5.*t296;
t398 = Ixx5.*t304;
t399 = Ixx6.*t307;
t400 = Ixy5.*t304;
t401 = Ixy6.*t307;
t402 = Ixz5.*t304;
t406 = Izx5.*t303;
t407 = Izx6.*t303;
t408 = Izy5.*t303;
t409 = Izy6.*t303;
t410 = Izz5.*t303;
t411 = Izz6.*t303;
t412 = Lxcm6.*t307;
t434 = Ixx6.*t315;
t436 = Ixy6.*t315;
t438 = Ixz6.*t315;
t440 = Iyx6.*t314;
t442 = Iyy6.*t314;
t443 = Izx5.*t310;
t444 = Izx6.*t310;
t445 = Izy5.*t310;
t446 = Izy6.*t310;
t447 = Izz5.*t310;
t450 = Lycm6.*t314;
t452 = Lz5.*t310;
t455 = Lzcm6.*t310;
t484 = Iyx6.*t322;
t485 = Iyy6.*t322;
t486 = Iyz6.*t322;
t499 = -t183;
t500 = -t184;
t501 = -t189;
t520 = -t252;
t536 = t13.*t304;
t540 = -t296;
t545 = -t310;
t550 = -t322;
t583 = t7.*t296;
t597 = t13.*t296;
t598 = t7.*t304;
t664 = Lxcm6.*t8.*t315;
t679 = Lycm6.*t8.*t322;
t700 = -t403;
t714 = -t435;
t719 = -t448;
t735 = -t482;
t736 = -t483;
t739 = -t487;
t777 = -t539;
t906 = -t745;
t907 = -t746;
t908 = -t747;
t914 = t5.*t638;
t915 = t5.*t639;
t941 = t62+t158;
t942 = t63+t160;
t943 = t70+t162;
t970 = -t931;
t971 = -t932;
t972 = -t840;
t973 = -t841;
t974 = t37.*t616;
t975 = -t847;
t976 = t37.*t621;
t977 = -t936;
t978 = -t872;
t979 = -t873;
t985 = -t889;
t986 = -t890;
t992 = -t951;
t993 = -t895;
t994 = -t896;
t1007 = t130+t304;
t1008 = t131+t303;
t1016 = -t956;
t1017 = -t957;
t1025 = -t1012;
t1028 = t37.*t882;
t1033 = t46+t91+t152;
t1034 = t37.*t918;
t1035 = -t1003;
t1037 = Lx3.*t1013;
t1040 = Lx3.*t1014;
t1045 = t5.*t1013;
t1046 = t11.*t1013;
t1047 = t5.*t1014;
t1048 = t11.*t1014;
t1049 = (t45.*t795)./2.0;
t1050 = (t49.*t796)./2.0;
t1051 = t312+t537;
t1064 = t159+t178+t207;
t1065 = t89+t211+t498;
t1066 = t150+t203+t256;
t1067 = t68+t205+t521;
t1094 = (t5.*t45.*t1059)./2.0;
t1095 = (t11.*t49.*t1058)./2.0;
t1130 = t103+t104+t153+t230+t231+t526+t527;
t1152 = t73+t102+t105+t229+t262+t416+t496+t532+t729+t741;
t1163 = t72+t168+t170+t191+t224+t395+t492+t523+t705+t727;
t1182 = t72+t186+t222+t413+t415+t494+t511+t525+t533+t535+t635+t637+t671+t672+t673+t682+t728+t834+t842+t859+t860+t861+t876+t878+t905+t966+t997;
t609 = Ixy6.*t583;
t622 = Ixx6.*t598;
t623 = Ixy6.*t598;
t625 = Iyy6.*t597;
t626 = Iyz6.*t597;
t632 = Lxcm6.*t598;
t643 = Iyx6.*t536;
t644 = Iyy6.*t536;
t646 = Lycm6.*t536;
t687 = -t392;
t688 = -t394;
t701 = -t412;
t715 = -t436;
t716 = -t443;
t717 = -t444;
t718 = -t447;
t720 = -t452;
out1 = ft_2({Ixx2,Ixx4,Ixx5,Ixx6,Ixy2,Ixy3,Ixy4,Ixy5,Ixy6,Ixz2,Ixz4,Ixz5,Ixz6,Iyx2,Iyx3,Iyx4,Iyx5,Iyx6,Iyy4,Iyy5,Iyy6,Iyz2,Iyz3,Iyz4,Iyz5,Iyz6,Izx2,Izx4,Izx5,Izx6,Izy2,Izy3,Izy4,Izy5,Izy6,Izz2,Izz5,Izz6,Lx2,Lxcm2,Lxcm3,Lxcm4,Lxcm5,Lxcm6,Lycm2,Lycm3,Lycm4,Lycm5,Lycm6,Lz4,Lz5,Lzcm2,Lzcm3,Lzcm4,Lzcm5,Lzcm6,m2,m3,m4,m5,m6,t10,t100,t1000,t1001,t1003,t1005,t1006,t1007,t1008,t1009,t101,t1010,t1015,t1016,t1017,t1018,t1019,t102,t1022,t1023,t1024,t1025,t1026,t1027,t1028,t1029,t1030,t1031,t1032,t1033,t1034,t1035,t1036,t1037,t1040,t1045,t1046,t1047,t1048,t1049,t1050,t1051,t1059,t1064,t1065,t1066,t1067,t107,t1070,t1074,t108,t109,t1094,t1095,t11,t110,t111,t112,t113,t1130,t114,t1152,t116,t1163,t1179,t1182,t12,t120,t122,t123,t124,t125,t127,t128,t129,t13,t131,t136,t137,t141,t142,t144,t145,t146,t147,t148,t149,t151,t154,t155,t156,t157,t161,t163,t164,t165,t166,t167,t169,t17,t171,t172,t175,t176,t177,t181,t182,t185,t186,t188,t190,t192,t193,t196,t198,t199,t2,t20,t200,t202,t204,t206,t210,t212,t213,t214,t215,t216,t217,t218,t219,t221,t222,t224,t227,t228,t232,t233,t235,t236,t237,t239,t240,t241,t242,t243,t244,t245,t246,t247,t248,t249,t250,t251,t253,t255,t257,t260,t262,t264,t27,t270,t271,t272,t273,t274,t276,t277,t278,t279,t28,t280,t281,t282,t283,t286,t288,t289,t29,t290,t291,t292,t293,t294,t295,t298,t299,t3,t30,t301,t302,t305,t306,t307,t31,t311,t313,t314,t315,t316,t32,t321,t324,t325,t328,t329,t330,t331,t332,t333,t334,t335,t336,t337,t338,t339,t340,t341,t342,t343,t344,t345,t346,t347,t348,t349,t350,t351,t354,t355,t356,t357,t358,t359,t36,t360,t362,t363,t364,t366,t367,t369,t37,t371,t372,t373,t374,t375,t376,t377,t379,t38,t382,t383,t384,t387,t389,t39,t390,t391,t393,t397,t398,t399,t4,t400,t401,t402,t404,t405,t406,t407,t408,t409,t410,t411,t414,t417,t418,t419,t422,t423,t425,t426,t427,t428,t429,t430,t431,t432,t433,t434,t437,t438,t439,t440,t441,t442,t445,t446,t449,t45,t450,t451,t453,t454,t455,t456,t457,t458,t459,t46,t460,t461,t467,t468,t469,t470,t472,t474,t475,t476,t477,t478,t479,t480,t481,t484,t485,t486,t488,t489,t49,t493,t495,t497,t499,t5,t50,t500,t501,t502,t503,t504,t505,t506,t507,t508,t509,t51,t510,t512,t513,t514,t515,t516,t517,t518,t519,t52,t520,t522,t524,t528,t529,t53,t530,t531,t534,t536,t54,t540,t542,t545,t549,t55,t550,t551,t553,t554,t556,t558,t56,t561,t562,t565,t568,t57,t570,t572,t573,t577,t578,t579,t58,t580,t581,t582,t585,t586,t587,t589,t59,t590,t591,t592,t593,t594,t595,t596,t597,t598,t6,t600,t601,t606,t607,t609,t61,t611,t612,t613,t614,t615,t616,t617,t618,t619,t620,t621,t622,t623,t625,t626,t627,t628,t629,t630,t631,t632,t633,t636,t638,t639,t640,t641,t642,t643,t644,t645,t646,t648,t650,t656,t657,t658,t659,t660,t661,t662,t663,t664,t665,t667,t668,t677,t678,t679,t680,t681,t683,t687,t688,t689,t69,t690,t691,t692,t693,t694,t695,t696,t697,t698,t699,t7,t700,t701,t703,t706,t707,t708,t709,t710,t711,t714,t715,t716,t717,t718,t719,t72,t720,t722,t723,t724,t726,t730,t731,t732,t733,t734,t735,t736,t739,t74,t740,t742,t743,t744,t746,t748,t749,t75,t750,t751,t753,t756,t759,t76,t760,t761,t762,t764,t765,t766,t767,t768,t769,t771,t773,t775,t777,t778,t779,t780,t782,t784,t785,t789,t79,t790,t792,t793,t794,t797,t799,t8,t801,t802,t803,t804,t805,t807,t810,t812,t814,t815,t817,t82,t821,t822,t823,t826,t827,t828,t831,t832,t835,t843,t844,t845,t846,t848,t849,t850,t852,t853,t854,t855,t856,t857,t858,t862,t863,t864,t865,t866,t867,t869,t870,t871,t874,t875,t877,t879,t880,t881,t882,t883,t884,t885,t886,t887,t888,t891,t893,t897,t898,t899,t9,t90,t900,t901,t902,t903,t904,t906,t907,t908,t909,t910,t911,t913,t914,t915,t916,t917,t918,t919,t92,t920,t921,t922,t923,t924,t925,t926,t928,t929,t93,t930,t931,t932,t934,t935,t938,t94,t941,t942,t943,t944,t945,t946,t947,t95,t953,t954,t955,t957,t958,t96,t961,t967,t968,t969,t97,t970,t971,t972,t973,t974,t975,t976,t977,t978,t979,t98,t980,t981,t983,t984,t985,t986,t987,t988,t989,t99,t990,t991,t992,t993,t994,t995,t996,t998,t999});
end
function out1 = ft_2(ct)
[Ixx2,Ixx4,Ixx5,Ixx6,Ixy2,Ixy3,Ixy4,Ixy5,Ixy6,Ixz2,Ixz4,Ixz5,Ixz6,Iyx2,Iyx3,Iyx4,Iyx5,Iyx6,Iyy4,Iyy5,Iyy6,Iyz2,Iyz3,Iyz4,Iyz5,Iyz6,Izx2,Izx4,Izx5,Izx6,Izy2,Izy3,Izy4,Izy5,Izy6,Izz2,Izz5,Izz6,Lx2,Lxcm2,Lxcm3,Lxcm4,Lxcm5,Lxcm6,Lycm2,Lycm3,Lycm4,Lycm5,Lycm6,Lz4,Lz5,Lzcm2,Lzcm3,Lzcm4,Lzcm5,Lzcm6,m2,m3,m4,m5,m6,t10,t100,t1000,t1001,t1003,t1005,t1006,t1007,t1008,t1009,t101,t1010,t1015,t1016,t1017,t1018,t1019,t102,t1022,t1023,t1024,t1025,t1026,t1027,t1028,t1029,t1030,t1031,t1032,t1033,t1034,t1035,t1036,t1037,t1040,t1045,t1046,t1047,t1048,t1049,t1050,t1051,t1059,t1064,t1065,t1066,t1067,t107,t1070,t1074,t108,t109,t1094,t1095,t11,t110,t111,t112,t113,t1130,t114,t1152,t116,t1163,t1179,t1182,t12,t120,t122,t123,t124,t125,t127,t128,t129,t13,t131,t136,t137,t141,t142,t144,t145,t146,t147,t148,t149,t151,t154,t155,t156,t157,t161,t163,t164,t165,t166,t167,t169,t17,t171,t172,t175,t176,t177,t181,t182,t185,t186,t188,t190,t192,t193,t196,t198,t199,t2,t20,t200,t202,t204,t206,t210,t212,t213,t214,t215,t216,t217,t218,t219,t221,t222,t224,t227,t228,t232,t233,t235,t236,t237,t239,t240,t241,t242,t243,t244,t245,t246,t247,t248,t249,t250,t251,t253,t255,t257,t260,t262,t264,t27,t270,t271,t272,t273,t274,t276,t277,t278,t279,t28,t280,t281,t282,t283,t286,t288,t289,t29,t290,t291,t292,t293,t294,t295,t298,t299,t3,t30,t301,t302,t305,t306,t307,t31,t311,t313,t314,t315,t316,t32,t321,t324,t325,t328,t329,t330,t331,t332,t333,t334,t335,t336,t337,t338,t339,t340,t341,t342,t343,t344,t345,t346,t347,t348,t349,t350,t351,t354,t355,t356,t357,t358,t359,t36,t360,t362,t363,t364,t366,t367,t369,t37,t371,t372,t373,t374,t375,t376,t377,t379,t38,t382,t383,t384,t387,t389,t39,t390,t391,t393,t397,t398,t399,t4,t400,t401,t402,t404,t405,t406,t407,t408,t409,t410,t411,t414,t417,t418,t419,t422,t423,t425,t426,t427,t428,t429,t430,t431,t432,t433,t434,t437,t438,t439,t440,t441,t442,t445,t446,t449,t45,t450,t451,t453,t454,t455,t456,t457,t458,t459,t46,t460,t461,t467,t468,t469,t470,t472,t474,t475,t476,t477,t478,t479,t480,t481,t484,t485,t486,t488,t489,t49,t493,t495,t497,t499,t5,t50,t500,t501,t502,t503,t504,t505,t506,t507,t508,t509,t51,t510,t512,t513,t514,t515,t516,t517,t518,t519,t52,t520,t522,t524,t528,t529,t53,t530,t531,t534,t536,t54,t540,t542,t545,t549,t55,t550,t551,t553,t554,t556,t558,t56,t561,t562,t565,t568,t57,t570,t572,t573,t577,t578,t579,t58,t580,t581,t582,t585,t586,t587,t589,t59,t590,t591,t592,t593,t594,t595,t596,t597,t598,t6,t600,t601,t606,t607,t609,t61,t611,t612,t613,t614,t615,t616,t617,t618,t619,t620,t621,t622,t623,t625,t626,t627,t628,t629,t630,t631,t632,t633,t636,t638,t639,t640,t641,t642,t643,t644,t645,t646,t648,t650,t656,t657,t658,t659,t660,t661,t662,t663,t664,t665,t667,t668,t677,t678,t679,t680,t681,t683,t687,t688,t689,t69,t690,t691,t692,t693,t694,t695,t696,t697,t698,t699,t7,t700,t701,t703,t706,t707,t708,t709,t710,t711,t714,t715,t716,t717,t718,t719,t72,t720,t722,t723,t724,t726,t730,t731,t732,t733,t734,t735,t736,t739,t74,t740,t742,t743,t744,t746,t748,t749,t75,t750,t751,t753,t756,t759,t76,t760,t761,t762,t764,t765,t766,t767,t768,t769,t771,t773,t775,t777,t778,t779,t780,t782,t784,t785,t789,t79,t790,t792,t793,t794,t797,t799,t8,t801,t802,t803,t804,t805,t807,t810,t812,t814,t815,t817,t82,t821,t822,t823,t826,t827,t828,t831,t832,t835,t843,t844,t845,t846,t848,t849,t850,t852,t853,t854,t855,t856,t857,t858,t862,t863,t864,t865,t866,t867,t869,t870,t871,t874,t875,t877,t879,t880,t881,t882,t883,t884,t885,t886,t887,t888,t891,t893,t897,t898,t899,t9,t90,t900,t901,t902,t903,t904,t906,t907,t908,t909,t910,t911,t913,t914,t915,t916,t917,t918,t919,t92,t920,t921,t922,t923,t924,t925,t926,t928,t929,t93,t930,t931,t932,t934,t935,t938,t94,t941,t942,t943,t944,t945,t946,t947,t95,t953,t954,t955,t957,t958,t96,t961,t967,t968,t969,t97,t970,t971,t972,t973,t974,t975,t976,t977,t978,t979,t98,t980,t981,t983,t984,t985,t986,t987,t988,t989,t99,t990,t991,t992,t993,t994,t995,t996,t998,t999] = ct{:};
t721 = -t455;
t737 = -t485;
t738 = -t486;
t818 = t7.*t540;
t838 = Iyx6.*t13.*t540;
t868 = -t664;
t1038 = t125+t545;
t1039 = t137+t540;
t1041 = Ixx5.*t1007;
t1042 = Ixz5.*t1007;
t1043 = t7.*t1007;
t1044 = t13.*t1007;
t1057 = -t1050;
t1060 = (t45.*t942)./2.0;
t1061 = (t49.*t941)./2.0;
t1062 = t306+t777;
t1068 = t56+t1046;
t1069 = t55+t1047;
t1079 = t313+t314+t536;
t1083 = -t12.*(t61-t1045);
t1085 = -t7.*(t50-t1048);
t1091 = t305+t550+t597;
t1092 = t307+t549+t598;
t1096 = (t45.*t1065)./2.0;
t1097 = t6.*(t61-t1045);
t1098 = (t49.*t1067)./2.0;
t1099 = t7.*(t50-t1048);
t1108 = (t5.*t49.*t1064)./2.0;
t1109 = (t11.*t45.*t1066)./2.0;
t1110 = t210+t215+t393+t408+t520;
t1113 = t204+t257+t400+t445+t499;
t1133 = t46+t1130;
t1162 = t90+t151+t221+t417+t418+t467+t468+t501+t528+t529;
t1177 = t74+t102+t219+t232+t260+t271+t453+t497+t633+t657+t730+t739+t874+t880;
t1178 = t72+t169+t186+t222+t414+t493+t524+t534+t613+t636+t706+t719+t858+t877;
t836 = Ixx6.*t818;
t837 = Ixz6.*t818;
t839 = -t632;
t1052 = Izx5.*t1038;
t1053 = Izx6.*t1038;
t1054 = Izy6.*t1038;
t1055 = Izz5.*t1038;
t1056 = Izz6.*t1038;
t1073 = t12.*t1069;
t1075 = t7.*t1068;
t1076 = t6.*t1069;
t1077 = t13.*t1068;
t1078 = t313+t1044;
t1089 = Iyz6.*t1079;
t1090 = t311+t315+t818;
t1100 = Ixz6.*t1092;
t1101 = -Ixx6.*(t321-t1043);
t1106 = -t1096;
t1107 = -t1098;
t1111 = t212+t217+t253+t410+t688;
t1112 = t181+t202+t255+t398+t716;
t1116 = t213+t251+t406+t508+t687;
t1117 = t185+t206+t402+t522+t718;
t1121 = t1026+t1083;
t1125 = t1027+t1097;
t1131 = (t11.*t45.*t1113)./2.0;
t1132 = (t11.*t49.*t1110)./2.0;
t1148 = t182+t399+t439+t440+t622+t643+t717+t735;
t1149 = t401+t441+t442+t446+t500+t623+t644+t736;
t1156 = t216+t404+t409+t609+t625+t714+t715+t737;
t1164 = t46+t1162;
t1180 = t102+t192+t219+t233+t260+t270+t272+t419+t451+t454+t656+t658+t679+t683+t695+t731+t835+t862+t868+t875+t879+t881+t911+t967+t969;
t1084 = -t1076;
t1086 = Iyx6.*t1078;
t1087 = Iyy6.*t1078;
t1088 = Iyz6.*t1078;
t1105 = -t1089;
t1114 = t1029+t1073;
t1115 = t255+t1041+t1052;
t1122 = t522+t1042+t1055;
t1123 = Lz5.*t1121;
t1124 = Lzcm6.*t1121;
t1128 = t13.*t1125;
t1129 = t7.*t1125;
t1134 = (t1007.*t1116)./2.0;
t1135 = (t1038.*t1111)./2.0;
t1136 = (t1039.*t1112)./2.0;
t1137 = (t1008.*t1117)./2.0;
t1146 = t218+t405+t411+t437+t438+t626+t738+t837;
t1155 = t214+t407+t433+t434+t484+t700+t836+t838;
t1169 = t69+t161+t188+t190+t449+t450+t488+t646+t701+t720+t721+t839;
t1170 = (t1090.*t1148)./2.0;
t1171 = (t1079.*t1156)./2.0;
t1172 = (t1091.*t1149)./2.0;
t1118 = t1030+t1084;
t1119 = Lz5.*t1114;
t1120 = Lzcm6.*t1114;
t1138 = -t1134;
t1139 = -t1135;
t1140 = -t1136;
t1141 = -t1137;
t1142 = t1077+t1129;
t1151 = t1053+t1086+t1101;
t1158 = -Lycm6.*(t1075-t1128);
t1159 = t1056+t1100+t1105;
t1165 = (t1038.*t1146)./2.0;
t1173 = -t1170;
t1174 = (t1092.*t1155)./2.0;
t1176 = t116+t1169;
t1126 = t7.*t1118;
t1127 = t13.*t1118;
t1150 = Lxcm6.*t1142;
t1166 = (t1008.*t1159)./2.0;
t1167 = -t1165;
t1175 = -t1174;
t1144 = Lxcm6.*(t1126-t13.*(t50-t1048));
t1147 = t1099+t1127;
t1157 = -t1150;
t1168 = -t1166;
t1153 = -t1144;
t1154 = Lycm6.*t1147;
t1183 = t72+t1006+t1037+t1123+t1124+t1157+t1158;
t1181 = t102+t1010+t1040+t1119+t1120+t1153+t1154;
et1 = (Ixy2.*t3.*t28)./2.0+(Iyx2.*t3.*t28)./2.0+(Iyz2.*t9.*t28)./2.0+(Izy2.*t9.*t28)./2.0+(Ixy3.*t3.*t4.*t28)./2.0+(Ixy3.*t3.*t4.*t29)./2.0-(Ixy4.*t3.*t4.*t28)./2.0-(Ixy4.*t3.*t4.*t29)./2.0-(Ixy3.*t9.*t10.*t28)./2.0-(Ixy3.*t9.*t10.*t29)./2.0+(Ixy4.*t9.*t10.*t28)./2.0+(Ixy4.*t9.*t10.*t29)./2.0+(Iyx3.*t3.*t4.*t28)./2.0+(Iyx3.*t3.*t4.*t29)./2.0-(Iyx4.*t3.*t4.*t28)./2.0-(Iyx4.*t3.*t4.*t29)./2.0-(Iyx3.*t9.*t10.*t28)./2.0-(Iyx3.*t9.*t10.*t29)./2.0+(Iyx4.*t9.*t10.*t28)./2.0+(Iyx4.*t9.*t10.*t29)./2.0+(Iyz3.*t3.*t10.*t28)./2.0+(Iyz3.*t4.*t9.*t28)./2.0+(Iyz3.*t3.*t10.*t29)./2.0+(Iyz3.*t4.*t9.*t29)./2.0;
et2 = (Izy3.*t3.*t10.*t28)./2.0+(Izy3.*t4.*t9.*t28)./2.0+(Izy3.*t3.*t10.*t29)./2.0+(Izy3.*t4.*t9.*t29)./2.0+Lycm3.*t9.*t28.*t53+Lycm3.*t9.*t29.*t53+Lycm3.*t9.*t28.*t148+Lycm3.*t9.*t29.*t148+t3.*t4.*t28.*t75+t3.*t4.*t28.*t76+t3.*t4.*t29.*t75+t3.*t4.*t29.*t76-t3.*t4.*t30.*t75-t3.*t4.*t30.*t76+t3.*t4.*t28.*t93+t3.*t4.*t29.*t93+t3.*t4.*t28.*t95+t3.*t4.*t28.*t96+t3.*t4.*t29.*t95+t3.*t4.*t29.*t96+t9.*t10.*t28.*t92-t9.*t10.*t28.*t93+t9.*t10.*t29.*t92-t9.*t10.*t29.*t93-t9.*t10.*t28.*t95+t3.*t4.*t28.*t108-t9.*t10.*t28.*t96-t9.*t10.*t29.*t95+t3.*t4.*t29.*t108-t9.*t10.*t29.*t96-t3.*t4.*t30.*t108+t9.*t10.*t28.*t98+t9.*t10.*t28.*t99+t9.*t10.*t29.*t98;
et3 = t9.*t10.*t29.*t99+t3.*t4.*t28.*t163+t3.*t4.*t28.*t164+t3.*t4.*t29.*t163+t3.*t4.*t28.*t165+t3.*t4.*t29.*t164+t3.*t4.*t29.*t165+t3.*t4.*t28.*t193+t3.*t4.*t29.*t193-t3.*t4.*t30.*t193-t3.*t4.*t32.*t193+t3.*t4.*t28.*t236+t3.*t4.*t28.*t237+t3.*t4.*t29.*t236+t3.*t4.*t29.*t237-t3.*t4.*t30.*t236-t3.*t4.*t30.*t237-t3.*t4.*t31.*t236-t3.*t4.*t32.*t237-t3.*t4.*t28.*t244-t3.*t4.*t29.*t244-t3.*t4.*t28.*t247+t3.*t4.*t31.*t244-t3.*t4.*t29.*t247-t3.*t4.*t32.*t244+t3.*t4.*t31.*t247-t3.*t4.*t32.*t247+t9.*t10.*t28.*t244+t9.*t10.*t29.*t244+t9.*t10.*t28.*t247-t9.*t10.*t31.*t244+t9.*t10.*t29.*t247+t9.*t10.*t32.*t244-t9.*t10.*t31.*t247;
et4 = t9.*t10.*t32.*t247+t3.*t4.*t28.*t277+t3.*t4.*t28.*t278+t3.*t4.*t29.*t277+t3.*t4.*t28.*t279+t3.*t4.*t29.*t278-t3.*t4.*t30.*t277+t3.*t4.*t29.*t279-t3.*t4.*t30.*t278-t3.*t4.*t31.*t277-t3.*t4.*t30.*t279-t3.*t4.*t31.*t278-t3.*t4.*t28.*t282-t3.*t4.*t31.*t279-t3.*t4.*t28.*t283-t3.*t4.*t29.*t282-t3.*t4.*t29.*t283+t3.*t4.*t31.*t282+t3.*t4.*t31.*t283-t3.*t4.*t32.*t282-t3.*t4.*t32.*t283+t9.*t10.*t28.*t282+t3.*t4.*t31.*t292+t9.*t10.*t28.*t283+t9.*t10.*t29.*t282+t9.*t10.*t29.*t283-t9.*t10.*t31.*t282+t3.*t4.*t31.*t295-t9.*t10.*t31.*t283+t9.*t10.*t32.*t282+t9.*t10.*t32.*t283+t3.*t4.*t31.*t299+t9.*t10.*t28.*t292+t3.*t4.*t31.*t302;
et5 = t9.*t10.*t29.*t292+t9.*t10.*t28.*t295+t9.*t10.*t29.*t295+t9.*t10.*t32.*t292+t9.*t10.*t28.*t299+t9.*t10.*t32.*t295+t9.*t10.*t29.*t299+t9.*t10.*t28.*t302+t9.*t10.*t29.*t302+t9.*t10.*t32.*t299+t9.*t10.*t32.*t302+t3.*t4.*t28.*t334+t3.*t4.*t29.*t334+t3.*t4.*t28.*t336+t3.*t4.*t29.*t336+t3.*t4.*t28.*t342+t3.*t4.*t29.*t342+t3.*t4.*t28.*t344+t3.*t4.*t29.*t344+t3.*t4.*t28.*t346+t3.*t4.*t29.*t346-t9.*t10.*t28.*t336-t9.*t10.*t29.*t336+t9.*t10.*t28.*t338+t9.*t10.*t28.*t339+t9.*t10.*t29.*t338+t9.*t10.*t28.*t340+t9.*t10.*t29.*t339+t9.*t10.*t29.*t340+t3.*t4.*t28.*t354.*2.0-t9.*t10.*t28.*t342-t3.*t4.*t28.*t355.*2.0+t3.*t4.*t29.*t354.*2.0-t9.*t10.*t29.*t342-t3.*t4.*t29.*t355.*2.0-t9.*t10.*t28.*t344;
et6 = -t9.*t10.*t29.*t344-t9.*t10.*t28.*t346-t9.*t10.*t29.*t346-t9.*t10.*t28.*t354.*2.0+t3.*t4.*t28.*t367+t9.*t10.*t28.*t355.*2.0-t9.*t10.*t29.*t354.*2.0+t3.*t4.*t29.*t367+t9.*t10.*t29.*t355.*2.0+t9.*t10.*t28.*t360+t9.*t10.*t29.*t360+t3.*t4.*t28.*t374+t9.*t10.*t28.*t362+t3.*t4.*t29.*t374+t9.*t10.*t29.*t362+t3.*t4.*t28.*t376+t3.*t4.*t29.*t376+t9.*t10.*t28.*t366-t9.*t10.*t28.*t367+t9.*t10.*t29.*t366-t9.*t10.*t29.*t367+t3.*t4.*t28.*t383.*2.0+t3.*t4.*t29.*t383.*2.0-t9.*t10.*t28.*t383.*2.0-t9.*t10.*t29.*t383.*2.0+t3.*t4.*t28.*t426+t3.*t4.*t29.*t426-t3.*t4.*t30.*t426-t3.*t4.*t31.*t426-t3.*t4.*t32.*t426+t3.*t4.*t28.*t458+t3.*t4.*t29.*t458+t3.*t4.*t28.*t461+t3.*t4.*t29.*t461;
et7 = t9.*t10.*t28.*t456+t9.*t10.*t29.*t456-t9.*t10.*t28.*t458+t9.*t10.*t28.*t459-t9.*t10.*t29.*t458+t9.*t10.*t29.*t459-t9.*t10.*t28.*t461+t3.*t4.*t30.*t472-t9.*t10.*t29.*t461+t3.*t4.*t31.*t472+t3.*t4.*t32.*t472+t3.*t4.*t28.*t593+t3.*t4.*t28.*t594+t3.*t4.*t29.*t593+t3.*t4.*t28.*t595+t3.*t4.*t29.*t594+t3.*t4.*t29.*t595+t3.*t4.*t28.*t600.*2.0+t3.*t4.*t28.*t601.*2.0+t3.*t4.*t29.*t600.*2.0+t3.*t4.*t29.*t601.*2.0-t9.*t10.*t28.*t600.*2.0-t9.*t10.*t28.*t601.*2.0-t9.*t10.*t29.*t600.*2.0+t3.*t4.*t28.*t614-t9.*t10.*t29.*t601.*2.0+t3.*t4.*t29.*t614+t3.*t4.*t28.*t616+t3.*t4.*t29.*t616+t3.*t4.*t28.*t618+t3.*t4.*t29.*t618+t3.*t4.*t28.*t648+t3.*t4.*t29.*t648+t3.*t4.*t28.*t650+t3.*t4.*t29.*t650;
et8 = -t9.*t10.*t28.*t648-t9.*t10.*t29.*t648-t9.*t10.*t28.*t650-t9.*t10.*t29.*t650+t9.*t10.*t28.*t667+t9.*t10.*t28.*t668+t9.*t10.*t29.*t667+t9.*t10.*t29.*t668+t3.*t4.*t28.*t698.*2.0+t3.*t4.*t28.*t699.*2.0+t3.*t4.*t29.*t698.*2.0+t3.*t4.*t29.*t699.*2.0-t9.*t10.*t28.*t698.*2.0-t9.*t10.*t28.*t699.*2.0-t9.*t10.*t29.*t698.*2.0-t9.*t10.*t29.*t699.*2.0+t3.*t4.*t28.*t722+t3.*t4.*t28.*t723+t3.*t4.*t29.*t722+t3.*t4.*t29.*t723+t3.*t4.*t28.*t733+t3.*t4.*t29.*t733-t3.*t4.*t28.*t746.*2.0-t3.*t4.*t29.*t746.*2.0+t3.*t4.*t28.*t749.*2.0+t3.*t4.*t28.*t750.*2.0+t3.*t4.*t29.*t749.*2.0+t3.*t4.*t28.*t751.*2.0+t3.*t4.*t29.*t750.*2.0+t3.*t4.*t29.*t751.*2.0+t9.*t10.*t28.*t746.*2.0+t3.*t4.*t28.*t759+t9.*t10.*t29.*t746.*2.0;
et9 = t3.*t4.*t29.*t759+t3.*t4.*t28.*t761-t9.*t10.*t28.*t749.*2.0+t3.*t4.*t29.*t761-t9.*t10.*t28.*t750.*2.0-t9.*t10.*t29.*t749.*2.0-t9.*t10.*t28.*t751.*2.0-t9.*t10.*t29.*t750.*2.0-t9.*t10.*t29.*t751.*2.0+t3.*t4.*t28.*t765+t3.*t4.*t29.*t765-t9.*t10.*t28.*t759-t9.*t10.*t29.*t759-t9.*t10.*t28.*t765+t9.*t10.*t28.*t766-t9.*t10.*t29.*t765+t9.*t10.*t29.*t766+t9.*t10.*t28.*t771+t9.*t10.*t29.*t771+t9.*t10.*t28.*t773+t9.*t10.*t29.*t773+t9.*t10.*t28.*t775+t9.*t10.*t29.*t775+t3.*t4.*t28.*t790+t3.*t4.*t29.*t790+t9.*t10.*t28.*t823+t9.*t10.*t29.*t823+t3.*t4.*t28.*t849+t3.*t4.*t29.*t849+t9.*t10.*t28.*t846+t9.*t10.*t29.*t846+t3.*t4.*t28.*t870+t3.*t4.*t28.*t871+t3.*t4.*t29.*t870+t3.*t4.*t29.*t871+t9.*t10.*t28.*t891;
et10 = t9.*t10.*t29.*t891+t9.*t10.*t28.*t893+t9.*t10.*t29.*t893+t3.*t4.*t28.*t909+t3.*t4.*t29.*t909+t3.*t4.*t28.*t919+t3.*t4.*t29.*t919+t3.*t4.*t28.*t921+t3.*t4.*t29.*t921+t3.*t4.*t28.*t923+t3.*t4.*t29.*t923+t3.*t4.*t28.*t925+t3.*t4.*t29.*t925+t9.*t10.*t28.*t931+t9.*t10.*t28.*t932+t9.*t10.*t29.*t931+t9.*t10.*t29.*t932+t3.*t4.*t28.*t954.*2.0+t3.*t4.*t29.*t954.*2.0-t3.*t4.*t28.*t957.*2.0-t3.*t4.*t29.*t957.*2.0-t9.*t10.*t28.*t954.*2.0-t9.*t10.*t29.*t954.*2.0+t9.*t10.*t28.*t957.*2.0+t9.*t10.*t29.*t957.*2.0+t3.*t4.*t28.*t974+t3.*t4.*t29.*t974+t3.*t4.*t28.*t987+t3.*t4.*t29.*t987+t3.*t4.*t28.*t989+t3.*t4.*t29.*t989+t3.*t4.*t28.*t1000+t3.*t4.*t29.*t1000+t9.*t10.*t28.*t1003+t9.*t10.*t29.*t1003+t3.*t4.*t28.*t1024+t3.*t4.*t29.*t1024;
et11 = t3.*t4.*t28.*t1035+t3.*t4.*t29.*t1035+Lx2.*Lycm3.*m3.*t3.*t28+Lxcm2.*Lycm2.*m2.*t3.*t28+Lycm2.*Lzcm2.*m2.*t9.*t28-(Ixy5.*t3.*t4.*t6.*t28)./2.0-(Ixy5.*t3.*t4.*t6.*t29)./2.0+(Ixy6.*t3.*t4.*t6.*t28)./2.0+(Ixy6.*t3.*t4.*t6.*t29)./2.0+(Ixy5.*t3.*t4.*t6.*t31)./2.0-(Ixy6.*t3.*t4.*t6.*t31)./2.0+(Ixy5.*t6.*t9.*t10.*t28)./2.0+(Ixy5.*t6.*t9.*t10.*t29)./2.0-(Ixy6.*t6.*t9.*t10.*t28)./2.0-(Ixy6.*t6.*t9.*t10.*t29)./2.0-(Ixy5.*t6.*t9.*t10.*t31)./2.0+(Ixy6.*t6.*t9.*t10.*t31)./2.0+Ixy4.*t3.*t4.*t28.*t36+Ixy4.*t3.*t4.*t29.*t36-Ixy4.*t9.*t10.*t28.*t36-Ixy4.*t9.*t10.*t29.*t36+(Ixz4.*t3.*t10.*t11.*t28)./2.0+(Ixz4.*t4.*t9.*t11.*t28)./2.0+(Ixz4.*t3.*t10.*t11.*t29)./2.0;
et12 = (Ixz4.*t4.*t9.*t11.*t29)./2.0-(Ixz5.*t3.*t10.*t11.*t28)./2.0-(Ixz5.*t4.*t9.*t11.*t28)./2.0-(Ixz4.*t3.*t10.*t11.*t30)./2.0-(Ixz4.*t4.*t9.*t11.*t30)./2.0-(Ixz5.*t3.*t10.*t11.*t29)./2.0-(Ixz5.*t4.*t9.*t11.*t29)./2.0+(Ixz5.*t3.*t10.*t11.*t30)./2.0+(Ixz5.*t4.*t9.*t11.*t30)./2.0-(Iyx5.*t3.*t4.*t6.*t28)./2.0-(Iyx5.*t3.*t4.*t6.*t29)./2.0+(Iyx6.*t3.*t4.*t6.*t28)./2.0+(Iyx6.*t3.*t4.*t6.*t29)./2.0+(Iyx5.*t3.*t4.*t6.*t31)./2.0-(Iyx6.*t3.*t4.*t6.*t31)./2.0+(Iyx5.*t6.*t9.*t10.*t28)./2.0+(Iyx5.*t6.*t9.*t10.*t29)./2.0-(Iyx6.*t6.*t9.*t10.*t28)./2.0-(Iyx6.*t6.*t9.*t10.*t29)./2.0-(Iyx5.*t6.*t9.*t10.*t31)./2.0;
et13 = (Iyx6.*t6.*t9.*t10.*t31)./2.0+Iyx4.*t3.*t4.*t28.*t36+Iyx4.*t3.*t4.*t29.*t36-Iyx4.*t9.*t10.*t28.*t36-Iyx4.*t9.*t10.*t29.*t36+(Iyz4.*t3.*t5.*t10.*t28)./2.0+(Iyz4.*t4.*t5.*t9.*t28)./2.0+(Iyz4.*t3.*t5.*t10.*t29)./2.0+(Iyz4.*t4.*t5.*t9.*t29)./2.0-(Iyz4.*t3.*t5.*t10.*t30)./2.0-(Iyz4.*t4.*t5.*t9.*t30)./2.0-(Iyz5.*t3.*t4.*t12.*t28)./2.0-(Iyz5.*t3.*t4.*t12.*t29)./2.0+(Iyz5.*t3.*t4.*t12.*t31)./2.0+(Iyz5.*t9.*t10.*t12.*t28)./2.0+(Iyz5.*t9.*t10.*t12.*t29)./2.0-(Iyz5.*t9.*t10.*t12.*t31)./2.0+(Izx4.*t3.*t10.*t11.*t28)./2.0+(Izx4.*t4.*t9.*t11.*t28)./2.0+(Izx4.*t3.*t10.*t11.*t29)./2.0+(Izx4.*t4.*t9.*t11.*t29)./2.0-(Izx5.*t3.*t10.*t11.*t28)./2.0;
et14 = Izx5.*t4.*t9.*t11.*t28.*(-1.0./2.0)-(Izx4.*t3.*t10.*t11.*t30)./2.0-(Izx4.*t4.*t9.*t11.*t30)./2.0-(Izx5.*t3.*t10.*t11.*t29)./2.0-(Izx5.*t4.*t9.*t11.*t29)./2.0+(Izx5.*t3.*t10.*t11.*t30)./2.0+(Izx5.*t4.*t9.*t11.*t30)./2.0+(Izy4.*t3.*t5.*t10.*t28)./2.0+(Izy4.*t4.*t5.*t9.*t28)./2.0+(Izy4.*t3.*t5.*t10.*t29)./2.0+(Izy4.*t4.*t5.*t9.*t29)./2.0-(Izy4.*t3.*t5.*t10.*t30)./2.0-(Izy4.*t4.*t5.*t9.*t30)./2.0-(Izy5.*t3.*t4.*t12.*t28)./2.0-(Izy5.*t3.*t4.*t12.*t29)./2.0+(Izy5.*t3.*t4.*t12.*t31)./2.0+(Izy5.*t9.*t10.*t12.*t28)./2.0+(Izy5.*t9.*t10.*t12.*t29)./2.0-(Izy5.*t9.*t10.*t12.*t31)./2.0+Lxcm4.*t9.*t11.*t28.*t54+Lxcm4.*t9.*t11.*t29.*t54;
et15 = -Lxcm4.*t9.*t11.*t30.*t54+Lxcm4.*t9.*t11.*t30.*t57+Lxcm4.*t9.*t11.*t28.*t145+Lxcm4.*t9.*t11.*t29.*t145+Lycm5.*t5.*t9.*t28.*t51+Lycm5.*t5.*t9.*t29.*t51+Lycm4.*t5.*t9.*t28.*t54-Lycm5.*t5.*t9.*t30.*t51+Lycm4.*t5.*t9.*t29.*t54-Lycm4.*t5.*t9.*t30.*t54+Lycm4.*t5.*t9.*t30.*t57+Lycm5.*t5.*t9.*t30.*t58+Lycm5.*t5.*t9.*t28.*t128+Lycm5.*t5.*t9.*t29.*t128-Lycm5.*t5.*t9.*t30.*t128+Lycm5.*t5.*t9.*t31.*t128+Lycm5.*t5.*t9.*t30.*t136+Lycm4.*t5.*t9.*t28.*t145+Lycm4.*t5.*t9.*t29.*t145+Lycm5.*t5.*t9.*t28.*t146+Lycm5.*t5.*t9.*t29.*t146+Lycm5.*t5.*t9.*t28.*t325+Lycm5.*t5.*t9.*t29.*t325+Lycm5.*t5.*t9.*t31.*t325+t3.*t10.*t11.*t28.*t79+t3.*t10.*t11.*t29.*t79-t3.*t10.*t11.*t30.*t79-t3.*t10.*t11.*t31.*t79+t3.*t10.*t11.*t28.*t94+t4.*t9.*t11.*t28.*t94+t3.*t10.*t11.*t29.*t94;
et16 = t4.*t9.*t11.*t29.*t94-t3.*t10.*t11.*t30.*t94-t4.*t9.*t11.*t30.*t94+t3.*t10.*t11.*t28.*t97+t4.*t9.*t11.*t28.*t97+t3.*t10.*t11.*t29.*t97+t4.*t9.*t11.*t29.*t97-t3.*t10.*t11.*t30.*t97-t4.*t9.*t11.*t30.*t97+t3.*t10.*t11.*t30.*t100+t4.*t9.*t11.*t30.*t100+t3.*t10.*t11.*t30.*t101+t4.*t9.*t11.*t30.*t101+t3.*t10.*t11.*t28.*t112+t3.*t10.*t11.*t28.*t113+t3.*t10.*t11.*t29.*t112+t3.*t10.*t11.*t28.*t114+t3.*t10.*t11.*t29.*t113-t3.*t10.*t11.*t30.*t112+t3.*t10.*t11.*t29.*t114-t3.*t10.*t11.*t30.*t113-t3.*t10.*t11.*t31.*t112-t3.*t10.*t11.*t30.*t114-t3.*t10.*t11.*t31.*t113-t3.*t10.*t11.*t31.*t114+t3.*t10.*t11.*t28.*t166+t4.*t9.*t11.*t28.*t166+t3.*t10.*t11.*t28.*t167+t3.*t10.*t11.*t29.*t166+t4.*t9.*t11.*t28.*t167;
et17 = t4.*t9.*t11.*t29.*t166+t3.*t10.*t11.*t29.*t167+t4.*t9.*t11.*t29.*t167+t9.*t10.*t28.*t37.*t164+t9.*t10.*t28.*t37.*t165+t9.*t10.*t29.*t37.*t164+t3.*t10.*t11.*t28.*t198+t9.*t10.*t29.*t37.*t165+t3.*t10.*t11.*t29.*t198-t3.*t10.*t11.*t30.*t198-t3.*t10.*t11.*t31.*t198-t3.*t10.*t11.*t32.*t198+t3.*t10.*t11.*t30.*t241+t3.*t10.*t11.*t31.*t241+t3.*t10.*t11.*t32.*t241+t3.*t10.*t11.*t28.*t335+t3.*t10.*t11.*t29.*t335+t3.*t10.*t11.*t30.*t337+t4.*t9.*t11.*t30.*t337+t3.*t10.*t11.*t28.*t343+t3.*t10.*t11.*t30.*t341+t4.*t9.*t11.*t28.*t343+t4.*t9.*t11.*t30.*t341+t3.*t10.*t11.*t29.*t343+t4.*t9.*t11.*t29.*t343+t3.*t10.*t11.*t28.*t345-t3.*t10.*t11.*t30.*t343+t4.*t9.*t11.*t28.*t345-t4.*t9.*t11.*t30.*t343+t3.*t10.*t11.*t29.*t345+t4.*t9.*t11.*t29.*t345;
et18 = t3.*t10.*t11.*t28.*t347-t3.*t10.*t11.*t30.*t345+t4.*t9.*t11.*t28.*t347-t4.*t9.*t11.*t30.*t345+t3.*t10.*t11.*t29.*t347+t4.*t9.*t11.*t29.*t347-t3.*t10.*t11.*t30.*t347-t4.*t9.*t11.*t30.*t347+t3.*t10.*t11.*t28.*t356.*2.0+t4.*t9.*t11.*t28.*t356.*2.0+t3.*t10.*t11.*t28.*t357.*2.0+t3.*t10.*t11.*t29.*t356.*2.0+t4.*t9.*t11.*t28.*t357.*2.0+t4.*t9.*t11.*t29.*t356.*2.0+t3.*t10.*t11.*t29.*t357.*2.0-t3.*t10.*t11.*t30.*t356.*2.0+t4.*t9.*t11.*t29.*t357.*2.0-t4.*t9.*t11.*t30.*t356.*2.0-t3.*t10.*t11.*t30.*t357.*2.0-t4.*t9.*t11.*t30.*t357.*2.0+t3.*t10.*t11.*t28.*t363+t4.*t9.*t11.*t28.*t363+t3.*t10.*t11.*t29.*t363+t4.*t9.*t11.*t29.*t363-t3.*t10.*t11.*t30.*t363-t4.*t9.*t11.*t30.*t363+t3.*t10.*t11.*t30.*t369+t4.*t9.*t11.*t30.*t369;
et19 = t3.*t4.*t28.*t38.*t355.*4.0+t3.*t4.*t29.*t38.*t355.*4.0-t3.*t10.*t11.*t28.*t382.*2.0-t4.*t9.*t11.*t28.*t382.*2.0-t3.*t10.*t11.*t29.*t382.*2.0-t4.*t9.*t11.*t29.*t382.*2.0-t3.*t10.*t11.*t28.*t384.*2.0+t3.*t10.*t11.*t30.*t382.*2.0-t4.*t9.*t11.*t28.*t384.*2.0+t4.*t9.*t11.*t30.*t382.*2.0-t3.*t10.*t11.*t29.*t384.*2.0-t4.*t9.*t11.*t29.*t384.*2.0+t3.*t10.*t11.*t30.*t384.*2.0+t4.*t9.*t11.*t30.*t384.*2.0-t9.*t10.*t28.*t38.*t355.*4.0-t9.*t10.*t29.*t38.*t355.*4.0+t3.*t10.*t11.*t28.*t457+t4.*t9.*t11.*t28.*t457+t3.*t10.*t11.*t29.*t457+t4.*t9.*t11.*t29.*t457-t3.*t10.*t11.*t30.*t457-t4.*t9.*t11.*t30.*t457+t3.*t10.*t11.*t28.*t460+t4.*t9.*t11.*t28.*t460+t3.*t10.*t11.*t29.*t460+t4.*t9.*t11.*t29.*t460-t3.*t10.*t11.*t30.*t460;
et20 = -t4.*t9.*t11.*t30.*t460+t3.*t10.*t11.*t28.*t514+t3.*t10.*t11.*t29.*t514+t3.*t10.*t11.*t28.*t592+t4.*t9.*t11.*t28.*t592+t3.*t10.*t11.*t29.*t592+t4.*t9.*t11.*t29.*t592+t3.*t10.*t11.*t28.*t596+t4.*t9.*t11.*t28.*t596+t3.*t10.*t11.*t29.*t596+t4.*t9.*t11.*t29.*t596+t3.*t10.*t11.*t28.*t620+t4.*t9.*t11.*t28.*t620+t3.*t10.*t11.*t29.*t620+t4.*t9.*t11.*t29.*t620+t9.*t10.*t28.*t38.*t593+t9.*t10.*t29.*t38.*t593+t9.*t10.*t28.*t38.*t618+t9.*t10.*t29.*t38.*t618-t6.*t9.*t10.*t28.*t661.*2.0-t6.*t9.*t10.*t29.*t661.*2.0-t6.*t9.*t10.*t28.*t663.*2.0-t6.*t9.*t10.*t29.*t663.*2.0+t3.*t10.*t11.*t30.*t762+t4.*t9.*t11.*t30.*t762+t3.*t10.*t11.*t28.*t768+t4.*t9.*t11.*t28.*t768+t3.*t10.*t11.*t29.*t768+t4.*t9.*t11.*t29.*t768+t3.*t10.*t11.*t28.*t917+t4.*t9.*t11.*t28.*t917;
et21 = t3.*t10.*t11.*t29.*t917+t4.*t9.*t11.*t29.*t917+t3.*t10.*t11.*t30.*t38.*t596+t4.*t9.*t11.*t30.*t38.*t596+t9.*t10.*t28.*t37.*t38.*t593+t9.*t10.*t29.*t37.*t38.*t593+Lx2.*Lxcm4.*m4.*t3.*t11.*t28-Lx2.*Lxcm4.*m4.*t3.*t11.*t30+Lx2.*Lycm4.*m4.*t3.*t5.*t28-Lx2.*Lycm4.*m4.*t3.*t5.*t30+Lx2.*Lycm5.*m5.*t3.*t5.*t28-Lx2.*Lycm5.*m5.*t3.*t5.*t30+Lxcm3.*Lycm3.*m3.*t3.*t4.*t28+Lxcm3.*Lycm3.*m3.*t3.*t4.*t29-Lxcm4.*Lycm4.*m4.*t3.*t4.*t28-Lxcm4.*Lycm4.*m4.*t3.*t4.*t29+Lxcm4.*Lycm4.*m4.*t9.*t10.*t28+Lxcm4.*Lycm4.*m4.*t9.*t10.*t29+Lycm3.*Lzcm3.*m3.*t3.*t10.*t28+Lycm3.*Lzcm3.*m3.*t3.*t10.*t29-(Ixy5.*t3.*t5.*t10.*t12.*t28)./2.0-(Ixy5.*t4.*t5.*t9.*t12.*t28)./2.0-(Ixy5.*t3.*t5.*t10.*t12.*t29)./2.0-(Ixy5.*t4.*t5.*t9.*t12.*t29)./2.0;
et22 = (Ixy6.*t3.*t5.*t10.*t12.*t28)./2.0+(Ixy6.*t4.*t5.*t9.*t12.*t28)./2.0+(Ixy5.*t3.*t5.*t10.*t12.*t30)./2.0+(Ixy5.*t4.*t5.*t9.*t12.*t30)./2.0+(Ixy6.*t3.*t5.*t10.*t12.*t29)./2.0+(Ixy6.*t4.*t5.*t9.*t12.*t29)./2.0-(Ixy5.*t3.*t5.*t10.*t12.*t31)./2.0-(Ixy5.*t4.*t5.*t9.*t12.*t31)./2.0-(Ixy6.*t3.*t5.*t10.*t12.*t30)./2.0-(Ixy6.*t4.*t5.*t9.*t12.*t30)./2.0+(Ixy6.*t3.*t5.*t10.*t12.*t31)./2.0+(Ixy6.*t4.*t5.*t9.*t12.*t31)./2.0+Ixy5.*t3.*t4.*t6.*t28.*t36+Ixy5.*t3.*t4.*t6.*t29.*t36-Ixy6.*t3.*t4.*t6.*t28.*t36-Ixy6.*t3.*t4.*t6.*t29.*t36-Ixy6.*t3.*t4.*t6.*t28.*t38-Ixy6.*t3.*t4.*t6.*t29.*t38+Ixy6.*t3.*t4.*t6.*t31.*t38-Ixy5.*t6.*t9.*t10.*t28.*t36-Ixy5.*t6.*t9.*t10.*t29.*t36;
et23 = Ixy6.*t6.*t9.*t10.*t28.*t36+Ixy6.*t6.*t9.*t10.*t29.*t36+Ixy6.*t6.*t9.*t10.*t28.*t38+Ixy6.*t6.*t9.*t10.*t29.*t38-Ixy6.*t6.*t9.*t10.*t31.*t38-(Ixz6.*t3.*t7.*t10.*t11.*t28)./2.0-(Ixz6.*t4.*t7.*t9.*t11.*t28)./2.0-(Ixz6.*t3.*t4.*t12.*t13.*t28)./2.0-(Ixz6.*t3.*t7.*t10.*t11.*t29)./2.0-(Ixz6.*t4.*t7.*t9.*t11.*t29)./2.0-(Ixz6.*t3.*t4.*t12.*t13.*t29)./2.0+(Ixz6.*t3.*t7.*t10.*t11.*t30)./2.0+(Ixz6.*t4.*t7.*t9.*t11.*t30)./2.0-(Ixz6.*t3.*t7.*t10.*t11.*t32)./2.0-(Ixz6.*t4.*t7.*t9.*t11.*t32)./2.0-(Ixz6.*t3.*t4.*t12.*t13.*t32)./2.0-(Ixz6.*t9.*t10.*t12.*t13.*t31)./2.0+Ixz5.*t3.*t10.*t11.*t28.*t37+Ixz5.*t4.*t9.*t11.*t28.*t37+Ixz5.*t3.*t10.*t11.*t29.*t37+Ixz5.*t4.*t9.*t11.*t29.*t37;
et24 = -Ixz5.*t3.*t10.*t11.*t30.*t37-Ixz5.*t4.*t9.*t11.*t30.*t37-(Iyx5.*t3.*t5.*t10.*t12.*t28)./2.0-(Iyx5.*t4.*t5.*t9.*t12.*t28)./2.0-(Iyx5.*t3.*t5.*t10.*t12.*t29)./2.0-(Iyx5.*t4.*t5.*t9.*t12.*t29)./2.0+(Iyx6.*t3.*t5.*t10.*t12.*t28)./2.0+(Iyx6.*t4.*t5.*t9.*t12.*t28)./2.0+(Iyx5.*t3.*t5.*t10.*t12.*t30)./2.0+(Iyx5.*t4.*t5.*t9.*t12.*t30)./2.0+(Iyx6.*t3.*t5.*t10.*t12.*t29)./2.0+(Iyx6.*t4.*t5.*t9.*t12.*t29)./2.0-(Iyx5.*t3.*t5.*t10.*t12.*t31)./2.0-(Iyx5.*t4.*t5.*t9.*t12.*t31)./2.0-(Iyx6.*t3.*t5.*t10.*t12.*t30)./2.0-(Iyx6.*t4.*t5.*t9.*t12.*t30)./2.0+(Iyx6.*t3.*t5.*t10.*t12.*t31)./2.0+(Iyx6.*t4.*t5.*t9.*t12.*t31)./2.0+Iyx5.*t3.*t4.*t6.*t28.*t36+Iyx5.*t3.*t4.*t6.*t29.*t36;
et25 = -Iyx6.*t3.*t4.*t6.*t28.*t36-Iyx6.*t3.*t4.*t6.*t29.*t36-Iyx6.*t3.*t4.*t6.*t28.*t38-Iyx6.*t3.*t4.*t6.*t29.*t38+Iyx6.*t3.*t4.*t6.*t31.*t38-Iyx5.*t6.*t9.*t10.*t28.*t36-Iyx5.*t6.*t9.*t10.*t29.*t36+Iyx6.*t6.*t9.*t10.*t28.*t36+Iyx6.*t6.*t9.*t10.*t29.*t36+Iyx6.*t6.*t9.*t10.*t28.*t38+Iyx6.*t6.*t9.*t10.*t29.*t38-Iyx6.*t6.*t9.*t10.*t31.*t38+(Iyz5.*t3.*t5.*t6.*t10.*t28)./2.0+(Iyz5.*t4.*t5.*t6.*t9.*t28)./2.0+(Iyz5.*t3.*t5.*t6.*t10.*t29)./2.0+(Iyz5.*t4.*t5.*t6.*t9.*t29)./2.0-(Iyz5.*t3.*t5.*t6.*t10.*t30)./2.0-(Iyz5.*t4.*t5.*t6.*t9.*t30)./2.0+(Iyz5.*t3.*t5.*t6.*t10.*t31)./2.0+(Iyz5.*t4.*t5.*t6.*t9.*t31)./2.0-(Iyz6.*t3.*t4.*t7.*t12.*t28)./2.0;
et26 = Iyz6.*t3.*t4.*t7.*t12.*t29.*(-1.0./2.0)-(Iyz6.*t3.*t4.*t7.*t12.*t32)./2.0+(Iyz6.*t3.*t10.*t11.*t13.*t28)./2.0+(Iyz6.*t4.*t9.*t11.*t13.*t28)./2.0+(Iyz6.*t3.*t10.*t11.*t13.*t29)./2.0+(Iyz6.*t4.*t9.*t11.*t13.*t29)./2.0-(Iyz6.*t3.*t10.*t11.*t13.*t30)./2.0-(Iyz6.*t4.*t9.*t11.*t13.*t30)./2.0+(Iyz6.*t3.*t10.*t11.*t13.*t32)./2.0+(Iyz6.*t4.*t9.*t11.*t13.*t32)./2.0-(Iyz6.*t7.*t9.*t10.*t12.*t31)./2.0+Iyz5.*t3.*t4.*t12.*t28.*t36+Iyz5.*t3.*t4.*t12.*t29.*t36-Iyz5.*t9.*t10.*t12.*t28.*t36-Iyz5.*t9.*t10.*t12.*t29.*t36-(Izx6.*t3.*t7.*t10.*t11.*t28)./2.0-(Izx6.*t4.*t7.*t9.*t11.*t28)./2.0-(Izx6.*t3.*t4.*t12.*t13.*t28)./2.0-(Izx6.*t3.*t7.*t10.*t11.*t29)./2.0;
et27 = Izx6.*t4.*t7.*t9.*t11.*t29.*(-1.0./2.0)-(Izx6.*t3.*t4.*t12.*t13.*t29)./2.0+(Izx6.*t3.*t7.*t10.*t11.*t30)./2.0+(Izx6.*t4.*t7.*t9.*t11.*t30)./2.0-(Izx6.*t3.*t7.*t10.*t11.*t32)./2.0-(Izx6.*t4.*t7.*t9.*t11.*t32)./2.0-(Izx6.*t3.*t4.*t12.*t13.*t32)./2.0-(Izx6.*t9.*t10.*t12.*t13.*t31)./2.0+Izx5.*t3.*t10.*t11.*t28.*t37+Izx5.*t4.*t9.*t11.*t28.*t37+Izx5.*t3.*t10.*t11.*t29.*t37+Izx5.*t4.*t9.*t11.*t29.*t37-Izx5.*t3.*t10.*t11.*t30.*t37-Izx5.*t4.*t9.*t11.*t30.*t37+(Izy5.*t3.*t5.*t6.*t10.*t28)./2.0+(Izy5.*t4.*t5.*t6.*t9.*t28)./2.0+(Izy5.*t3.*t5.*t6.*t10.*t29)./2.0+(Izy5.*t4.*t5.*t6.*t9.*t29)./2.0-(Izy5.*t3.*t5.*t6.*t10.*t30)./2.0-(Izy5.*t4.*t5.*t6.*t9.*t30)./2.0;
et28 = (Izy5.*t3.*t5.*t6.*t10.*t31)./2.0+(Izy5.*t4.*t5.*t6.*t9.*t31)./2.0-(Izy6.*t3.*t4.*t7.*t12.*t28)./2.0-(Izy6.*t3.*t4.*t7.*t12.*t29)./2.0-(Izy6.*t3.*t4.*t7.*t12.*t32)./2.0+(Izy6.*t3.*t10.*t11.*t13.*t28)./2.0+(Izy6.*t4.*t9.*t11.*t13.*t28)./2.0+(Izy6.*t3.*t10.*t11.*t13.*t29)./2.0+(Izy6.*t4.*t9.*t11.*t13.*t29)./2.0-(Izy6.*t3.*t10.*t11.*t13.*t30)./2.0-(Izy6.*t4.*t9.*t11.*t13.*t30)./2.0+(Izy6.*t3.*t10.*t11.*t13.*t32)./2.0+(Izy6.*t4.*t9.*t11.*t13.*t32)./2.0-(Izy6.*t7.*t9.*t10.*t12.*t31)./2.0+Izy5.*t3.*t4.*t12.*t28.*t36+Izy5.*t3.*t4.*t12.*t29.*t36-Izy5.*t9.*t10.*t12.*t28.*t36-Izy5.*t9.*t10.*t12.*t29.*t36+Lxcm5.*t6.*t9.*t11.*t28.*t51+Lxcm5.*t6.*t9.*t11.*t29.*t51;
et29 = -Lxcm5.*t6.*t9.*t11.*t30.*t51-Lxcm5.*t6.*t9.*t11.*t31.*t51+Lxcm6.*t5.*t9.*t13.*t28.*t52+Lxcm6.*t5.*t9.*t13.*t29.*t52-Lxcm6.*t5.*t9.*t13.*t30.*t52-Lxcm6.*t5.*t9.*t13.*t32.*t52+Lxcm5.*t6.*t9.*t11.*t30.*t58+Lxcm5.*t6.*t9.*t11.*t31.*t58+Lxcm6.*t5.*t9.*t13.*t30.*t59+Lxcm6.*t5.*t9.*t13.*t32.*t59+Lxcm6.*t5.*t9.*t13.*t28.*t127+Lxcm6.*t5.*t9.*t13.*t29.*t127+Lxcm6.*t5.*t9.*t13.*t28.*t129-Lxcm6.*t5.*t9.*t13.*t30.*t127+Lxcm6.*t5.*t9.*t13.*t29.*t129+Lxcm6.*t5.*t9.*t13.*t31.*t127-Lxcm6.*t5.*t9.*t13.*t30.*t129-Lxcm6.*t5.*t9.*t13.*t32.*t127+Lxcm6.*t5.*t9.*t13.*t31.*t129-Lxcm6.*t5.*t9.*t13.*t32.*t129+Lxcm5.*t6.*t9.*t11.*t28.*t146+Lxcm5.*t6.*t9.*t11.*t29.*t146+Lxcm6.*t5.*t9.*t13.*t28.*t147+Lxcm6.*t5.*t9.*t13.*t29.*t147+Lxcm6.*t5.*t9.*t13.*t28.*t316.*2.0+Lxcm6.*t5.*t9.*t13.*t29.*t316.*2.0;
et30 = Lycm6.*t5.*t7.*t9.*t28.*t52+Lycm6.*t5.*t7.*t9.*t29.*t52-Lycm6.*t5.*t7.*t9.*t30.*t52-Lycm6.*t5.*t7.*t9.*t32.*t52+Lycm6.*t5.*t7.*t9.*t30.*t59+Lycm6.*t5.*t7.*t9.*t32.*t59+Lycm6.*t5.*t7.*t9.*t28.*t127+Lycm6.*t5.*t7.*t9.*t29.*t127+Lycm6.*t5.*t7.*t9.*t28.*t129-Lycm6.*t5.*t7.*t9.*t30.*t127+Lycm6.*t5.*t7.*t9.*t29.*t129+Lycm6.*t5.*t7.*t9.*t31.*t127-Lycm6.*t5.*t7.*t9.*t30.*t129-Lycm6.*t5.*t7.*t9.*t32.*t127+Lycm6.*t5.*t7.*t9.*t31.*t129-Lycm6.*t5.*t7.*t9.*t32.*t129+Lycm6.*t5.*t7.*t9.*t28.*t147+Lycm6.*t5.*t7.*t9.*t29.*t147+Lz5.*t9.*t11.*t12.*t28.*t52+Lz5.*t9.*t11.*t12.*t29.*t52-Lz5.*t9.*t11.*t12.*t30.*t52-Lz5.*t9.*t11.*t12.*t31.*t52+Lz5.*t9.*t11.*t12.*t30.*t59+Lz5.*t9.*t11.*t12.*t31.*t59+Lz5.*t9.*t11.*t12.*t28.*t147+Lz5.*t9.*t11.*t12.*t29.*t147;
et31 = Lzcm5.*t9.*t11.*t12.*t28.*t51+Lzcm5.*t9.*t11.*t12.*t29.*t51-Lzcm5.*t9.*t11.*t12.*t30.*t51+Lzcm6.*t9.*t11.*t12.*t28.*t52-Lzcm5.*t9.*t11.*t12.*t31.*t51+Lzcm6.*t9.*t11.*t12.*t29.*t52-Lzcm6.*t9.*t11.*t12.*t30.*t52-Lzcm6.*t9.*t11.*t12.*t31.*t52+Lzcm5.*t9.*t11.*t12.*t30.*t58+Lzcm5.*t9.*t11.*t12.*t31.*t58+Lzcm6.*t9.*t11.*t12.*t30.*t59+Lzcm6.*t9.*t11.*t12.*t31.*t59+Lzcm6.*t9.*t11.*t12.*t28.*t127.*2.0+Lzcm6.*t9.*t11.*t12.*t29.*t127.*2.0-Lzcm6.*t9.*t11.*t12.*t30.*t127.*2.0+Lzcm5.*t9.*t11.*t12.*t28.*t146+Lzcm5.*t9.*t11.*t12.*t29.*t146+Lzcm6.*t9.*t11.*t12.*t28.*t147+Lzcm6.*t9.*t11.*t12.*t29.*t147+Lx2.*Lxcm5.*m5.*t3.*t6.*t11.*t28-Lx2.*Lxcm5.*m5.*t3.*t6.*t11.*t30-Lx2.*Lxcm5.*m5.*t3.*t6.*t11.*t31+Lx2.*Lxcm6.*m6.*t3.*t5.*t13.*t28-Lx2.*Lxcm6.*m6.*t3.*t5.*t13.*t30;
et32 = -Lx2.*Lxcm6.*m6.*t3.*t5.*t13.*t32+Lx2.*Lycm6.*m6.*t3.*t5.*t7.*t28-Lx2.*Lycm6.*m6.*t3.*t5.*t7.*t30-Lx2.*Lycm6.*m6.*t3.*t5.*t7.*t32-Lxcm5.*Lycm5.*m5.*t3.*t4.*t6.*t28-Lxcm5.*Lycm5.*m5.*t3.*t4.*t6.*t29+Lxcm5.*Lycm5.*m5.*t3.*t4.*t6.*t31+Lxcm6.*Lycm6.*m6.*t3.*t4.*t6.*t28+Lxcm6.*Lycm6.*m6.*t3.*t4.*t6.*t29-Lxcm6.*Lycm6.*m6.*t3.*t4.*t6.*t31+Lxcm5.*Lycm5.*m5.*t6.*t9.*t10.*t28+Lxcm5.*Lycm5.*m5.*t6.*t9.*t10.*t29-Lxcm5.*Lycm5.*m5.*t6.*t9.*t10.*t31-Lxcm6.*Lycm6.*m6.*t6.*t9.*t10.*t28-Lxcm6.*Lycm6.*m6.*t6.*t9.*t10.*t29+Lxcm6.*Lycm6.*m6.*t6.*t9.*t10.*t31+Lxcm4.*Lycm4.*m4.*t3.*t4.*t28.*t36.*2.0+Lxcm4.*Lycm4.*m4.*t3.*t4.*t29.*t36.*2.0-Lxcm4.*Lycm4.*m4.*t9.*t10.*t28.*t36.*2.0-Lxcm4.*Lycm4.*m4.*t9.*t10.*t29.*t36.*2.0+Lx2.*Lz5.*m6.*t3.*t11.*t12.*t28;
et33 = -Lx2.*Lz5.*m6.*t3.*t11.*t12.*t30-Lx2.*Lz5.*m6.*t3.*t11.*t12.*t31+Lx2.*Lzcm5.*m5.*t3.*t11.*t12.*t28-Lx2.*Lzcm5.*m5.*t3.*t11.*t12.*t30+Lx2.*Lzcm6.*m6.*t3.*t11.*t12.*t28-Lx2.*Lzcm5.*m5.*t3.*t11.*t12.*t31-Lx2.*Lzcm6.*m6.*t3.*t11.*t12.*t30-Lx2.*Lzcm6.*m6.*t3.*t11.*t12.*t31+Lxcm4.*Lzcm4.*m4.*t3.*t10.*t11.*t28+Lxcm4.*Lzcm4.*m4.*t3.*t10.*t11.*t29-Lxcm4.*Lzcm4.*m4.*t3.*t10.*t11.*t30-Lxcm5.*Lzcm5.*m5.*t3.*t10.*t11.*t28-Lxcm5.*Lzcm5.*m5.*t4.*t9.*t11.*t28-Lxcm5.*Lzcm5.*m5.*t3.*t10.*t11.*t29-Lxcm5.*Lzcm5.*m5.*t4.*t9.*t11.*t29+Lxcm5.*Lzcm5.*m5.*t3.*t10.*t11.*t30+Lxcm5.*Lzcm5.*m5.*t4.*t9.*t11.*t30+Lycm5.*Lz4.*m5.*t3.*t5.*t10.*t28+Lycm5.*Lz4.*m5.*t3.*t5.*t10.*t29-Lycm5.*Lz4.*m5.*t3.*t5.*t10.*t30+Lycm4.*Lzcm4.*m4.*t3.*t5.*t10.*t28+Lycm4.*Lzcm4.*m4.*t3.*t5.*t10.*t29;
et34 = -Lycm4.*Lzcm4.*m4.*t3.*t5.*t10.*t30-Lycm5.*Lzcm5.*m5.*t3.*t4.*t12.*t28-Lycm5.*Lzcm5.*m5.*t3.*t4.*t12.*t29+Lycm5.*Lzcm5.*m5.*t3.*t4.*t12.*t31+Lycm5.*Lzcm5.*m5.*t9.*t10.*t12.*t28+Lycm5.*Lzcm5.*m5.*t9.*t10.*t12.*t29-Lycm5.*Lzcm5.*m5.*t9.*t10.*t12.*t31+Ixx6.*t3.*t4.*t6.*t7.*t13.*t28+Ixx6.*t3.*t4.*t6.*t7.*t13.*t29-Ixx6.*t3.*t4.*t6.*t7.*t13.*t31-Ixx6.*t6.*t7.*t9.*t10.*t13.*t28-Ixx6.*t6.*t7.*t9.*t10.*t13.*t29+Ixx6.*t6.*t7.*t9.*t10.*t13.*t31-Ixy6.*t3.*t5.*t10.*t12.*t28.*t38-Ixy6.*t4.*t5.*t9.*t12.*t28.*t38-Ixy6.*t3.*t5.*t10.*t12.*t29.*t38-Ixy6.*t4.*t5.*t9.*t12.*t29.*t38+Ixy6.*t3.*t5.*t10.*t12.*t30.*t38+Ixy6.*t4.*t5.*t9.*t12.*t30.*t38-Ixy6.*t3.*t5.*t10.*t12.*t31.*t38-Ixy6.*t4.*t5.*t9.*t12.*t31.*t38;
et35 = (Ixz6.*t3.*t5.*t6.*t10.*t13.*t28)./2.0+(Ixz6.*t4.*t5.*t6.*t9.*t13.*t28)./2.0+(Ixz6.*t3.*t5.*t6.*t10.*t13.*t29)./2.0+(Ixz6.*t4.*t5.*t6.*t9.*t13.*t29)./2.0-(Ixz6.*t3.*t5.*t6.*t10.*t13.*t30)./2.0-(Ixz6.*t4.*t5.*t6.*t9.*t13.*t30)./2.0+(Ixz6.*t3.*t5.*t6.*t10.*t13.*t31)./2.0+(Ixz6.*t4.*t5.*t6.*t9.*t13.*t31)./2.0-(Ixz6.*t3.*t5.*t6.*t10.*t13.*t32)./2.0-(Ixz6.*t4.*t5.*t6.*t9.*t13.*t32)./2.0+Ixz6.*t3.*t4.*t12.*t13.*t28.*t36+Ixz6.*t3.*t7.*t10.*t11.*t28.*t37+Ixz6.*t4.*t7.*t9.*t11.*t28.*t37+Ixz6.*t3.*t4.*t12.*t13.*t29.*t36+Ixz6.*t3.*t7.*t10.*t11.*t29.*t37+Ixz6.*t4.*t7.*t9.*t11.*t29.*t37-Ixz6.*t3.*t7.*t10.*t11.*t30.*t37-Ixz6.*t4.*t7.*t9.*t11.*t30.*t37-Ixz6.*t9.*t10.*t12.*t13.*t28.*t36;
et36 = -Ixz6.*t9.*t10.*t12.*t13.*t29.*t36-Iyx6.*t3.*t5.*t10.*t12.*t28.*t38-Iyx6.*t4.*t5.*t9.*t12.*t28.*t38-Iyx6.*t3.*t5.*t10.*t12.*t29.*t38-Iyx6.*t4.*t5.*t9.*t12.*t29.*t38+Iyx6.*t3.*t5.*t10.*t12.*t30.*t38+Iyx6.*t4.*t5.*t9.*t12.*t30.*t38-Iyx6.*t3.*t5.*t10.*t12.*t31.*t38-Iyx6.*t4.*t5.*t9.*t12.*t31.*t38-Iyy6.*t3.*t4.*t6.*t7.*t13.*t28-Iyy6.*t3.*t4.*t6.*t7.*t13.*t29+Iyy6.*t3.*t4.*t6.*t7.*t13.*t31+Iyy6.*t6.*t7.*t9.*t10.*t13.*t28+Iyy6.*t6.*t7.*t9.*t10.*t13.*t29-Iyy6.*t6.*t7.*t9.*t10.*t13.*t31+(Iyz6.*t3.*t5.*t6.*t7.*t10.*t28)./2.0+(Iyz6.*t4.*t5.*t6.*t7.*t9.*t28)./2.0+(Iyz6.*t3.*t5.*t6.*t7.*t10.*t29)./2.0+(Iyz6.*t4.*t5.*t6.*t7.*t9.*t29)./2.0-(Iyz6.*t3.*t5.*t6.*t7.*t10.*t30)./2.0;
et37 = Iyz6.*t4.*t5.*t6.*t7.*t9.*t30.*(-1.0./2.0)+(Iyz6.*t3.*t5.*t6.*t7.*t10.*t31)./2.0+(Iyz6.*t4.*t5.*t6.*t7.*t9.*t31)./2.0-(Iyz6.*t3.*t5.*t6.*t7.*t10.*t32)./2.0-(Iyz6.*t4.*t5.*t6.*t7.*t9.*t32)./2.0+Iyz6.*t3.*t4.*t7.*t12.*t28.*t36+Iyz6.*t3.*t4.*t7.*t12.*t29.*t36-Iyz6.*t3.*t10.*t11.*t13.*t28.*t37-Iyz6.*t4.*t9.*t11.*t13.*t28.*t37-Iyz6.*t7.*t9.*t10.*t12.*t28.*t36-Iyz6.*t3.*t10.*t11.*t13.*t29.*t37-Iyz6.*t4.*t9.*t11.*t13.*t29.*t37-Iyz6.*t7.*t9.*t10.*t12.*t29.*t36+Iyz6.*t3.*t10.*t11.*t13.*t30.*t37+Iyz6.*t4.*t9.*t11.*t13.*t30.*t37+(Izx6.*t3.*t5.*t6.*t10.*t13.*t28)./2.0+(Izx6.*t4.*t5.*t6.*t9.*t13.*t28)./2.0+(Izx6.*t3.*t5.*t6.*t10.*t13.*t29)./2.0+(Izx6.*t4.*t5.*t6.*t9.*t13.*t29)./2.0;
et38 = Izx6.*t3.*t5.*t6.*t10.*t13.*t30.*(-1.0./2.0)-(Izx6.*t4.*t5.*t6.*t9.*t13.*t30)./2.0+(Izx6.*t3.*t5.*t6.*t10.*t13.*t31)./2.0+(Izx6.*t4.*t5.*t6.*t9.*t13.*t31)./2.0-(Izx6.*t3.*t5.*t6.*t10.*t13.*t32)./2.0-(Izx6.*t4.*t5.*t6.*t9.*t13.*t32)./2.0+Izx6.*t3.*t4.*t12.*t13.*t28.*t36+Izx6.*t3.*t7.*t10.*t11.*t28.*t37+Izx6.*t4.*t7.*t9.*t11.*t28.*t37+Izx6.*t3.*t4.*t12.*t13.*t29.*t36+Izx6.*t3.*t7.*t10.*t11.*t29.*t37+Izx6.*t4.*t7.*t9.*t11.*t29.*t37-Izx6.*t3.*t7.*t10.*t11.*t30.*t37-Izx6.*t4.*t7.*t9.*t11.*t30.*t37-Izx6.*t9.*t10.*t12.*t13.*t28.*t36-Izx6.*t9.*t10.*t12.*t13.*t29.*t36+(Izy6.*t3.*t5.*t6.*t7.*t10.*t28)./2.0+(Izy6.*t4.*t5.*t6.*t7.*t9.*t28)./2.0+(Izy6.*t3.*t5.*t6.*t7.*t10.*t29)./2.0;
et39 = (Izy6.*t4.*t5.*t6.*t7.*t9.*t29)./2.0-(Izy6.*t3.*t5.*t6.*t7.*t10.*t30)./2.0-(Izy6.*t4.*t5.*t6.*t7.*t9.*t30)./2.0+(Izy6.*t3.*t5.*t6.*t7.*t10.*t31)./2.0+(Izy6.*t4.*t5.*t6.*t7.*t9.*t31)./2.0-(Izy6.*t3.*t5.*t6.*t7.*t10.*t32)./2.0-(Izy6.*t4.*t5.*t6.*t7.*t9.*t32)./2.0+Izy6.*t3.*t4.*t7.*t12.*t28.*t36+Izy6.*t3.*t4.*t7.*t12.*t29.*t36-Izy6.*t3.*t10.*t11.*t13.*t28.*t37-Izy6.*t4.*t9.*t11.*t13.*t28.*t37-Izy6.*t7.*t9.*t10.*t12.*t28.*t36-Izy6.*t3.*t10.*t11.*t13.*t29.*t37-Izy6.*t4.*t9.*t11.*t13.*t29.*t37-Izy6.*t7.*t9.*t10.*t12.*t29.*t36+Izy6.*t3.*t10.*t11.*t13.*t30.*t37+Izy6.*t4.*t9.*t11.*t13.*t30.*t37+Lxcm6.*t6.*t7.*t9.*t11.*t28.*t52+Lxcm6.*t6.*t7.*t9.*t11.*t29.*t52-Lxcm6.*t6.*t7.*t9.*t11.*t30.*t52;
et40 = -Lxcm6.*t6.*t7.*t9.*t11.*t31.*t52-Lxcm6.*t6.*t7.*t9.*t11.*t32.*t52+Lxcm6.*t6.*t7.*t9.*t11.*t30.*t59+Lxcm6.*t6.*t7.*t9.*t11.*t31.*t59+Lxcm6.*t6.*t7.*t9.*t11.*t32.*t59+Lxcm6.*t6.*t7.*t9.*t11.*t28.*t147+Lxcm6.*t6.*t7.*t9.*t11.*t29.*t147+Lxcm6.*t5.*t9.*t13.*t28.*t37.*t316.*2.0+Lxcm6.*t5.*t9.*t13.*t29.*t37.*t316.*2.0-Lycm6.*t6.*t9.*t11.*t13.*t28.*t52-Lycm6.*t6.*t9.*t11.*t13.*t29.*t52+Lycm6.*t6.*t9.*t11.*t13.*t30.*t52+Lycm6.*t6.*t9.*t11.*t13.*t31.*t52+Lycm6.*t6.*t9.*t11.*t13.*t32.*t52+Lycm6.*t6.*t9.*t11.*t13.*t28.*t59+Lycm6.*t6.*t9.*t11.*t13.*t29.*t59+Lycm6.*t6.*t9.*t11.*t13.*t30.*t147+Lycm6.*t6.*t9.*t11.*t13.*t31.*t147+Lycm6.*t6.*t9.*t11.*t13.*t32.*t147-t6.*t9.*t10.*t11.*t12.*t28.*t82.*2.0-t6.*t9.*t10.*t11.*t12.*t29.*t82.*2.0+t3.*t6.*t7.*t10.*t13.*t28.*t276.*2.0+t4.*t6.*t7.*t9.*t13.*t28.*t276.*2.0;
et41 = t3.*t6.*t7.*t10.*t13.*t29.*t276.*2.0+t4.*t6.*t7.*t9.*t13.*t29.*t276.*2.0-t3.*t6.*t7.*t10.*t13.*t30.*t276.*2.0-t4.*t6.*t7.*t9.*t13.*t30.*t276.*2.0+Lx2.*Lxcm6.*m6.*t3.*t6.*t7.*t11.*t28-Lx2.*Lxcm6.*m6.*t3.*t6.*t7.*t11.*t30-Lx2.*Lxcm6.*m6.*t3.*t6.*t7.*t11.*t31-Lx2.*Lxcm6.*m6.*t3.*t6.*t7.*t11.*t32-Lx2.*Lycm6.*m6.*t3.*t6.*t11.*t13.*t28+Lx2.*Lycm6.*m6.*t3.*t6.*t11.*t13.*t30+Lx2.*Lycm6.*m6.*t3.*t6.*t11.*t13.*t31+Lx2.*Lycm6.*m6.*t3.*t6.*t11.*t13.*t32-Lxcm5.*Lycm5.*m5.*t3.*t5.*t10.*t12.*t28-Lxcm5.*Lycm5.*m5.*t3.*t5.*t10.*t12.*t29+Lxcm5.*Lycm5.*m5.*t3.*t5.*t10.*t12.*t30-Lxcm5.*Lycm5.*m5.*t3.*t5.*t10.*t12.*t31+Lxcm6.*Lycm6.*m6.*t3.*t5.*t10.*t12.*t28+Lxcm6.*Lycm6.*m6.*t4.*t5.*t9.*t12.*t28+Lxcm6.*Lycm6.*m6.*t3.*t5.*t10.*t12.*t29+Lxcm6.*Lycm6.*m6.*t4.*t5.*t9.*t12.*t29;
et42 = -Lxcm6.*Lycm6.*m6.*t3.*t5.*t10.*t12.*t30-Lxcm6.*Lycm6.*m6.*t4.*t5.*t9.*t12.*t30+Lxcm6.*Lycm6.*m6.*t3.*t5.*t10.*t12.*t31+Lxcm6.*Lycm6.*m6.*t4.*t5.*t9.*t12.*t31-Lxcm6.*Lycm6.*m6.*t3.*t4.*t6.*t28.*t38.*2.0-Lxcm6.*Lycm6.*m6.*t3.*t4.*t6.*t29.*t38.*2.0+Lxcm6.*Lycm6.*m6.*t3.*t4.*t6.*t31.*t38.*2.0+Lxcm6.*Lycm6.*m6.*t6.*t9.*t10.*t28.*t38.*2.0+Lxcm6.*Lycm6.*m6.*t6.*t9.*t10.*t29.*t38.*2.0-Lxcm6.*Lycm6.*m6.*t6.*t9.*t10.*t31.*t38.*2.0+Lxcm6.*Lz4.*m6.*t3.*t5.*t10.*t13.*t28+Lxcm6.*Lz4.*m6.*t3.*t5.*t10.*t13.*t29-Lxcm6.*Lz5.*m6.*t3.*t7.*t10.*t11.*t28-Lxcm6.*Lz5.*m6.*t4.*t7.*t9.*t11.*t28-Lxcm6.*Lz4.*m6.*t3.*t5.*t10.*t13.*t30-Lxcm6.*Lz5.*m6.*t3.*t7.*t10.*t11.*t29-Lxcm6.*Lz5.*m6.*t4.*t7.*t9.*t11.*t29+Lxcm6.*Lz5.*m6.*t3.*t7.*t10.*t11.*t30+Lxcm6.*Lz5.*m6.*t4.*t7.*t9.*t11.*t30;
et43 = -Lxcm6.*Lz4.*m6.*t3.*t5.*t10.*t13.*t32-Lxcm6.*Lz5.*m6.*t3.*t7.*t10.*t11.*t32-Lxcm6.*Lz5.*m6.*t4.*t7.*t9.*t11.*t32-Lxcm6.*Lzcm6.*m6.*t3.*t7.*t10.*t11.*t28-Lxcm6.*Lzcm6.*m6.*t4.*t7.*t9.*t11.*t28-Lxcm6.*Lzcm6.*m6.*t3.*t7.*t10.*t11.*t29-Lxcm6.*Lzcm6.*m6.*t4.*t7.*t9.*t11.*t29+Lxcm6.*Lzcm6.*m6.*t3.*t7.*t10.*t11.*t30+Lxcm6.*Lzcm6.*m6.*t4.*t7.*t9.*t11.*t30-Lxcm6.*Lzcm6.*m6.*t3.*t7.*t10.*t11.*t32-Lxcm6.*Lzcm6.*m6.*t4.*t7.*t9.*t11.*t32+Lxcm5.*Lzcm5.*m5.*t3.*t10.*t11.*t28.*t37.*2.0+Lxcm5.*Lzcm5.*m5.*t4.*t9.*t11.*t28.*t37.*2.0+Lxcm5.*Lzcm5.*m5.*t3.*t10.*t11.*t29.*t37.*2.0+Lxcm5.*Lzcm5.*m5.*t4.*t9.*t11.*t29.*t37.*2.0-Lxcm5.*Lzcm5.*m5.*t3.*t10.*t11.*t30.*t37.*2.0-Lxcm5.*Lzcm5.*m5.*t4.*t9.*t11.*t30.*t37.*2.0+Lycm6.*Lz4.*m6.*t3.*t5.*t7.*t10.*t28+Lycm6.*Lz4.*m6.*t3.*t5.*t7.*t10.*t29;
et44 = -Lycm6.*Lz4.*m6.*t3.*t5.*t7.*t10.*t30-Lycm6.*Lz4.*m6.*t3.*t5.*t7.*t10.*t32+Lycm6.*Lz5.*m6.*t3.*t10.*t11.*t13.*t28+Lycm6.*Lz5.*m6.*t4.*t9.*t11.*t13.*t28+Lycm6.*Lz5.*m6.*t3.*t10.*t11.*t13.*t29+Lycm6.*Lz5.*m6.*t4.*t9.*t11.*t13.*t29-Lycm6.*Lz5.*m6.*t3.*t10.*t11.*t13.*t30-Lycm6.*Lz5.*m6.*t4.*t9.*t11.*t13.*t30+Lycm6.*Lz5.*m6.*t3.*t10.*t11.*t13.*t32+Lycm6.*Lz5.*m6.*t4.*t9.*t11.*t13.*t32+Lycm5.*Lzcm5.*m5.*t3.*t5.*t6.*t10.*t28+Lycm5.*Lzcm5.*m5.*t3.*t5.*t6.*t10.*t29-Lycm5.*Lzcm5.*m5.*t3.*t5.*t6.*t10.*t30+Lycm5.*Lzcm5.*m5.*t3.*t5.*t6.*t10.*t31+Lycm6.*Lzcm6.*m6.*t3.*t10.*t11.*t13.*t28+Lycm6.*Lzcm6.*m6.*t4.*t9.*t11.*t13.*t28+Lycm6.*Lzcm6.*m6.*t3.*t10.*t11.*t13.*t29+Lycm6.*Lzcm6.*m6.*t4.*t9.*t11.*t13.*t29-Lycm6.*Lzcm6.*m6.*t3.*t10.*t11.*t13.*t30-Lycm6.*Lzcm6.*m6.*t4.*t9.*t11.*t13.*t30;
et45 = Lycm6.*Lzcm6.*m6.*t3.*t10.*t11.*t13.*t32+Lycm6.*Lzcm6.*m6.*t4.*t9.*t11.*t13.*t32-Lz5.*Lzcm6.*m6.*t5.*t9.*t10.*t11.*t28.*2.0-Lz5.*Lzcm6.*m6.*t5.*t9.*t10.*t11.*t29.*2.0+Ixx6.*t3.*t5.*t7.*t10.*t12.*t13.*t28+Ixx6.*t4.*t5.*t7.*t9.*t12.*t13.*t28+Ixx6.*t3.*t5.*t7.*t10.*t12.*t13.*t29+Ixx6.*t4.*t5.*t7.*t9.*t12.*t13.*t29-Ixx6.*t3.*t5.*t7.*t10.*t12.*t13.*t30-Ixx6.*t4.*t5.*t7.*t9.*t12.*t13.*t30+Ixx6.*t3.*t5.*t7.*t10.*t12.*t13.*t31+Ixx6.*t4.*t5.*t7.*t9.*t12.*t13.*t31-Iyy6.*t3.*t5.*t7.*t10.*t12.*t13.*t28-Iyy6.*t4.*t5.*t7.*t9.*t12.*t13.*t28-Iyy6.*t3.*t5.*t7.*t10.*t12.*t13.*t29-Iyy6.*t4.*t5.*t7.*t9.*t12.*t13.*t29+Iyy6.*t3.*t5.*t7.*t10.*t12.*t13.*t30+Iyy6.*t4.*t5.*t7.*t9.*t12.*t13.*t30-Iyy6.*t3.*t5.*t7.*t10.*t12.*t13.*t31-Iyy6.*t4.*t5.*t7.*t9.*t12.*t13.*t31;
et46 = Lxcm6.*t3.*t5.*t7.*t11.*t12.*t28.*t127.*2.0+Lxcm6.*t3.*t5.*t7.*t11.*t12.*t29.*t127.*2.0+Lxcm6.*t3.*t5.*t7.*t11.*t12.*t28.*t129.*2.0+Lxcm6.*t3.*t5.*t7.*t11.*t12.*t29.*t129.*2.0-Lycm6.*t3.*t5.*t11.*t12.*t13.*t28.*t127.*2.0-Lycm6.*t3.*t5.*t11.*t12.*t13.*t29.*t127.*2.0-Lycm6.*t3.*t5.*t11.*t12.*t13.*t28.*t129.*2.0-Lycm6.*t3.*t5.*t11.*t12.*t13.*t29.*t129.*2.0-m6.*t3.*t4.*t6.*t7.*t13.*t17.*t28-m6.*t3.*t4.*t6.*t7.*t13.*t17.*t29+m6.*t3.*t4.*t6.*t7.*t13.*t17.*t31+m6.*t3.*t4.*t6.*t7.*t13.*t20.*t28+m6.*t3.*t4.*t6.*t7.*t13.*t20.*t29-m6.*t3.*t4.*t6.*t7.*t13.*t20.*t31+m6.*t6.*t7.*t9.*t10.*t13.*t17.*t28+m6.*t6.*t7.*t9.*t10.*t13.*t17.*t29-m6.*t6.*t7.*t9.*t10.*t13.*t17.*t31-m6.*t6.*t7.*t9.*t10.*t13.*t20.*t28-m6.*t6.*t7.*t9.*t10.*t13.*t20.*t29;
et47 = m6.*t6.*t7.*t9.*t10.*t13.*t20.*t31-Lxcm6.*Lycm6.*m6.*t3.*t5.*t10.*t12.*t28.*t38.*2.0-Lxcm6.*Lycm6.*m6.*t4.*t5.*t9.*t12.*t28.*t38.*2.0-Lxcm6.*Lycm6.*m6.*t3.*t5.*t10.*t12.*t29.*t38.*2.0-Lxcm6.*Lycm6.*m6.*t4.*t5.*t9.*t12.*t29.*t38.*2.0+Lxcm6.*Lycm6.*m6.*t3.*t5.*t10.*t12.*t30.*t38.*2.0+Lxcm6.*Lycm6.*m6.*t4.*t5.*t9.*t12.*t30.*t38.*2.0-Lxcm6.*Lycm6.*m6.*t3.*t5.*t10.*t12.*t31.*t38.*2.0-Lxcm6.*Lycm6.*m6.*t4.*t5.*t9.*t12.*t31.*t38.*2.0+Lxcm6.*Lz5.*m6.*t3.*t5.*t6.*t10.*t13.*t28+Lxcm6.*Lz5.*m6.*t3.*t5.*t6.*t10.*t13.*t29-Lxcm6.*Lz5.*m6.*t3.*t5.*t6.*t10.*t13.*t30+Lxcm6.*Lz5.*m6.*t3.*t5.*t6.*t10.*t13.*t31-Lxcm6.*Lz5.*m6.*t3.*t5.*t6.*t10.*t13.*t32+Lxcm6.*Lzcm6.*m6.*t3.*t5.*t6.*t10.*t13.*t28+Lxcm6.*Lzcm6.*m6.*t3.*t5.*t6.*t10.*t13.*t29-Lxcm6.*Lzcm6.*m6.*t3.*t5.*t6.*t10.*t13.*t30+Lxcm6.*Lzcm6.*m6.*t3.*t5.*t6.*t10.*t13.*t31;
et48 = -Lxcm6.*Lzcm6.*m6.*t3.*t5.*t6.*t10.*t13.*t32+Lycm6.*Lz5.*m6.*t3.*t5.*t6.*t7.*t10.*t28+Lycm6.*Lz5.*m6.*t3.*t5.*t6.*t7.*t10.*t29-Lycm6.*Lz5.*m6.*t3.*t5.*t6.*t7.*t10.*t30+Lycm6.*Lz5.*m6.*t3.*t5.*t6.*t7.*t10.*t31-Lycm6.*Lz5.*m6.*t3.*t5.*t6.*t7.*t10.*t32+Lycm6.*Lzcm6.*m6.*t3.*t5.*t6.*t7.*t10.*t28+Lycm6.*Lzcm6.*m6.*t3.*t5.*t6.*t7.*t10.*t29-Lycm6.*Lzcm6.*m6.*t3.*t5.*t6.*t7.*t10.*t30+Lycm6.*Lzcm6.*m6.*t3.*t5.*t6.*t7.*t10.*t31-Lycm6.*Lzcm6.*m6.*t3.*t5.*t6.*t7.*t10.*t32-Lz5.*Lzcm6.*m6.*t3.*t6.*t10.*t11.*t12.*t30.*2.0-m6.*t3.*t5.*t7.*t10.*t12.*t13.*t17.*t28-m6.*t4.*t5.*t7.*t9.*t12.*t13.*t17.*t28-m6.*t3.*t5.*t7.*t10.*t12.*t13.*t17.*t29-m6.*t4.*t5.*t7.*t9.*t12.*t13.*t17.*t29+m6.*t3.*t5.*t7.*t10.*t12.*t13.*t17.*t30+m6.*t4.*t5.*t7.*t9.*t12.*t13.*t17.*t30;
et49 = -m6.*t3.*t5.*t7.*t10.*t12.*t13.*t17.*t31+m6.*t3.*t5.*t7.*t10.*t12.*t13.*t20.*t28-m6.*t4.*t5.*t7.*t9.*t12.*t13.*t17.*t31+m6.*t4.*t5.*t7.*t9.*t12.*t13.*t20.*t28+m6.*t3.*t5.*t7.*t10.*t12.*t13.*t20.*t29+m6.*t4.*t5.*t7.*t9.*t12.*t13.*t20.*t29-m6.*t3.*t5.*t7.*t10.*t12.*t13.*t20.*t30-m6.*t4.*t5.*t7.*t9.*t12.*t13.*t20.*t30+m6.*t3.*t5.*t7.*t10.*t12.*t13.*t20.*t31+m6.*t4.*t5.*t7.*t9.*t12.*t13.*t20.*t31-Lxcm6.*Lycm6.*m6.*t3.*t4.*t5.*t7.*t11.*t13.*t28.*2.0-Lxcm6.*Lycm6.*m6.*t3.*t4.*t5.*t7.*t11.*t13.*t29.*2.0;
et50 = t30.*(t82+t110+t111+t120+t122+t123+t124+t157+t171+t172+t199+t200+t227+t228+t240+t245+t276+t280+t288+t289+t290+t293+t298+t301+t350+t351+t358+t359+t372+t373+t390+t391-t422+t427+t428+t431+t469-t475-t476-t477+t478+t480+t489+t495+t504+t509+t510+t515+t516+t517+t518+t519+t531+t572+t573+t578+t581+t586+t590+t606+t607+t612+t638+t639+t659+t697+t711+t740+t748+t792+t801+t802+t803+t821+t822+t826+t845+t852+t853+t903+t904+t906+t938+t953+t968+t1016+Lx2.*t141+Lx2.*t142+Lx2.*t324)+t32.*(t240+t243+t246+t274+t280+t291+t294+t348+t349-t423+t427+t428+t431+t469+t470+t478+t480+t495+t506+t507+t513+t578+t581+t586+t590+t659+t697+t845);
et51 = -t31.*(t109+t154+t155+t156+t196+t239+t245+t248+t249+t250+t276+t290+t293+t298+t301+t358+t359+t397+t422+t423+t428+t431-t470+t475+t476+t477+t478+t480+t489+t530+t531+t578+t581+t586+t590+t638+t639+t640-t659+t710+t740+t792+t826+t938-Lx2.*t127-Lx2.*t128-Lx2.*t129+Lx2.*t136);
et52 = -t27.*(t1049+t1057+t1060+t1061+t1094+t1095+t1106+t1107+t1108+t1109+t1131+t1132+t1138+t1139+t1140+t1141+t1167+t1168+t1171+t1172+t1173+t1175+(t3.*(Ixx2.*t9+Izx2.*t3))./2.0+(t9.*(Ixx2.*t3-Izx2.*t9))./2.0+(t3.*(Ixz2.*t3-Izz2.*t9))./2.0-(t9.*(Ixz2.*t9+Izz2.*t3))./2.0-m3.*t2.*t1033.*t1074-m3.*t8.*t1033.*t1070-m4.*t8.*t1133.*t1152-m4.*t2.*t1133.*t1163-m5.*t2.*t1164.*t1178-m5.*t8.*t1164.*t1177+m6.*t2.*t1176.*t1182+m6.*t8.*t1176.*t1180+m2.*t2.*t542.*(-Lycm2.*t8+Lxcm2.*t2.*t3+Lzcm2.*t2.*t9)+m2.*t8.*t542.*(Lycm2.*t2+Lxcm2.*t3.*t8+Lzcm2.*t8.*t9))+Lx2.*t29.*t1179;
et53 = t32.*(t240+t243+t246+t274+t280+t291+t294+t348+t349+t427+t428+t431+t478+t480+t506+t507+t513+t578+t581+t586+t590+t697)-t27.*(t1049+t1057+t1060+t1061+t1094+t1095+t1106+t1107+t1108+t1109+t1131+t1132+t1138+t1139+t1140+t1141+t1167+t1168+t1171+t1172+t1173+t1175+m3.*t2.*t943.*t1074+m3.*t8.*t943.*t1070-m4.*t8.*t1130.*t1152-m4.*t2.*t1130.*t1163-m5.*t2.*t1162.*t1178-m5.*t8.*t1162.*t1177+m6.*t2.*t1169.*t1182+m6.*t8.*t1169.*t1180)-t31.*(t109+t154+t155+t156+t196+t239+t245+t248+t249+t250+t276+t290+t293+t298+t301+t358+t359+t397+t428+t431+t478+t480+t489+t530+t531+t578+t581+t586+t590+t638+t639+t710+t740+t792+t826+t938);
et54 = t30.*(t82+t110+t111+t120+t122+t123+t124+t157+t171+t172+t199+t200+t227+t228+t240+t245+t276+t280+t288+t289+t290+t293+t298+t301+t350+t351+t358+t359+t372+t373+t390+t391+t427+t428+t431+t478+t480+t489+t504+t509+t510+t515+t516+t517+t518+t519+t531+t572+t573+t578+t581+t586+t590+t606+t607+t612+t638+t639+t697+t711+t740+t748+t792+t801+t802+t803+t821+t822+t826+t852+t853+t903+t904+t906+t938+t953+t968+t1016)-Lx2.*t28.*t1179;
et55 = ((t321-t1043).*(-Ixx6.*t1051+Iyx6.*t1062+Izx6.*t11.*t137))./2.0+(t1051.*t1151)./2.0+(t45.*(Ixz4.*t11.*t49+Iyz4.*t5.*t49))./2.0+(t1062.*(t1054-t1087+Ixy6.*(t321-t1043)))./2.0-(t1007.*(-Ixx5.*t11.*t131+Iyx5.*t5.*t49+Izx5.*t11.*t137))./2.0+(t1038.*(Ixz5.*t11.*t131+Iyz5.*t5.*t49-Izz5.*t11.*t137))./2.0+(t1078.*(Ixy6.*t1051-Iyy6.*t1062+Izy6.*t11.*t137))./2.0+(t1038.*(Ixz6.*t1051+Iyz6.*t1062-Izz6.*t11.*t137))./2.0+m6.*t1181.*(Lycm6.*(t7.*t1069+t6.*t13.*(t50-t1048))+Lxcm6.*(t13.*t1069+t6.*t1085)-Lz5.*t12.*(t50-t1048)-Lzcm6.*t12.*(t50-t1048));
et56 = (t11.*t137.*(-t1056+t1088+Ixz6.*(t321-t1043)))./2.0+m5.*t1178.*(Lycm5.*t149+Lxcm5.*t6.*t56+Lzcm5.*t12.*t56+t3.*t4.*t74-t9.*t10.*t74+t3.*t4.*t232-t9.*t10.*t232+t3.*t4.*t271-t9.*t10.*t271)-m5.*t1177.*(-Lycm5.*t55+Lxcm5.*t6.*t50+Lzcm5.*t12.*t50+t9.*t10.*t107+t3.*t4.*t169+t9.*t10.*t264+t9.*t10.*t286+t3.*t4.*t524+t3.*t4.*t534)-(t5.*t49.*(t257+Ixy5.*t1007-Izy5.*t1038))./2.0+(t11.*t49.*(Ixy5.*t11.*t131-Iyy5.*t5.*t49+Izy5.*t11.*t137))./2.0+m6.*t1183.*(Lxcm6.*(t6.*t1075-t13.*(t61-t1045))-Lycm6.*(t6.*t1077+t7.*(t61-t1045))+Lz5.*t12.*t1068+Lzcm6.*t12.*t1068)+(t11.*t49.*t1059)./2.0;
et57 = t5.*t49.*t1066.*(-1.0./2.0)+(t11.*t131.*t1115)./2.0-(t11.*t137.*t1122)./2.0+(t5.*t49.*(Ixx4.*t11.*t49-Iyx4.*t5.*t49))./2.0+(t11.*t49.*(Ixy4.*t11.*t49-Iyy4.*t5.*t49))./2.0+m4.*(Lxcm4.*t1068-Lycm4.*(t61-t1045)).*(t72+t224+t1037-Lycm4.*t1068-Lxcm4.*(t61-t1045))+m4.*(Lycm4.*t1069-Lxcm4.*(t50-t1048)).*(t102+t262+t1040+Lxcm4.*t1069+Lycm4.*(t50-t1048));
et58 = t28.*(t75+t76+t93+t95+t96+t108+t163+t164+t165+t175+t193+t236+t237+t277+t278+t279+t328+t331+t334+t336+t342+t344+t346+t354+t367+t374+t376+t379+t383+t426+t458+t461+t551+t554+t558+t561+t562+t565+t593+t594+t595+t600+t601+t611+t614+t616+t618+t627+t645+t648+t650+t680+t681+t689+t691+t698+t699+t707+t708+t722+t723+t733+t749+t750+t751+t753+t759+t761+t765+t778+t779+t780+t782+t790+t827+t828+t831+t832+t843+t844+t849+t863+t864+t865+t870+t871+t884+t885+t907+t909+t916+t919+t921+t923+t925+t929+t930+t935+t954+t961+t970+t971+t974+t977+t987+t989+t1000+t1017+t1018+t1024+t1035+Lx2.*Lxcm4.*m4.*t4.*t11+Lx2.*Lycm4.*m4.*t4.*t5+Lx2.*Lycm5.*m5.*t4.*t5+Lx2.*Lxcm5.*m5.*t4.*t6.*t11+Lx2.*Lxcm6.*m6.*t4.*t5.*t13+Lx2.*Lycm6.*m6.*t4.*t5.*t7+Lx2.*Lz5.*m6.*t4.*t11.*t12+Lx2.*Lzcm5.*m5.*t4.*t11.*t12+Lx2.*Lzcm6.*m6.*t4.*t11.*t12+Lx2.*Lxcm6.*m6.*t4.*t6.*t7.*t11-Lx2.*Lycm6.*m6.*t4.*t6.*t11.*t13);
et59 = t29.*(t75+t76+t93+t95+t96+t108+t163+t164+t165+t175+t193+t236+t237+t277+t278+t279+t328+t331+t334+t336+t342+t344+t346+t354+t367+t374+t376+t379+t383+t426+t458+t461+t551+t554+t558+t561+t562+t565+t593+t594+t595+t600+t601+t611+t614+t616+t618+t627+t645+t648+t650+t680+t681+t689+t691+t698+t699+t707+t708+t722+t723+t733+t749+t750+t751+t753+t759+t761+t765+t778+t779+t780+t782+t790+t827+t828+t831+t832+t843+t844+t849+t863+t864+t865+t870+t871+t884+t885+t907+t909+t916+t919+t921+t923+t925+t929+t930+t935+t954+t961+t970+t971+t974+t977+t987+t989+t1000+t1017+t1018+t1024+t1035)+t27.*(et55+et56+et57);
et60 = t31.*(t244+t247+t282+t283+t292+t295+t299+t302+(Ixy5.*t6)./2.0-(Ixy6.*t6)./2.0+(Iyx5.*t6)./2.0-(Iyx6.*t6)./2.0+(Iyz5.*t12)./2.0+(Izy5.*t12)./2.0+Ixy6.*t6.*t38+Iyx6.*t6.*t38-Ixx6.*t6.*t7.*t13+Iyy6.*t6.*t7.*t13+Lxcm5.*Lycm5.*m5.*t6-Lxcm6.*Lycm6.*m6.*t6+Lycm5.*Lzcm5.*m5.*t12+Lxcm6.*Lycm6.*m6.*t6.*t38.*2.0+m6.*t6.*t7.*t13.*t17-m6.*t6.*t7.*t13.*t20)-t32.*(t244+t247+t282+t283+t292+t295+t299+t302);
et61 = (t1007.*t1122)./2.0-(t1038.*t1115)./2.0-(t1007.*(Ixx5.*t1038-Izx5.*t1007))./2.0-(t1038.*(Ixz5.*t1038-Izz5.*t1007))./2.0-(t1078.*(Izy6.*t1007+Ixy6.*t7.*t1038+Iyy6.*t13.*t1038))./2.0+(t1038.*(Izz6.*t1007-Ixz6.*t7.*t1038+Iyz6.*t13.*t1038))./2.0+((t321-t1043).*(-Izx6.*t1007+Ixx6.*t7.*t1038+Iyx6.*t13.*t1038))./2.0-(t1007.*(-t1056+t1088+Ixz6.*(t321-t1043)))./2.0+m6.*t1181.*(Lz5.*t1118+Lzcm6.*t1118+Lxcm6.*t7.*t1114-Lycm6.*t13.*t1114)+m6.*t1183.*(Lz5.*t1125+Lzcm6.*t1125+Lxcm6.*t7.*t1121-Lycm6.*t13.*t1121)+(t13.*t1038.*(t1054-t1087+Ixy6.*(t321-t1043)))./2.0-(t7.*t1038.*t1151)./2.0;
et62 = m5.*t1177.*(Lxcm5.*t12.*t55+Lxcm5.*t8.*t131-Lzcm5.*t6.*t55+Lzcm5.*t8.*t137+Lxcm5.*t3.*t4.*t12.*t56-Lxcm5.*t9.*t10.*t12.*t56-Lzcm5.*t3.*t4.*t6.*t56+Lzcm5.*t6.*t9.*t10.*t56)+m5.*t1178.*(Lxcm5.*t2.*t131+Lxcm5.*t12.*t149+Lzcm5.*t6.*t61+Lzcm5.*t2.*t137+Lxcm5.*t3.*t4.*t12.*t50+Lxcm5.*t9.*t10.*t12.*t144+Lzcm5.*t6.*t9.*t10.*t50+Lzcm5.*t3.*t4.*t6.*t144)-(t11.*t49.*(Ixy5.*t1038+Izy5.*t1007))./2.0;
et63 = -t32.*((Ixz6.*t7)./2.0-(Iyz6.*t13)./2.0+(Izx6.*t7)./2.0-(Izy6.*t13)./2.0+Lxcm6.*Lz5.*m6.*t7+Lxcm6.*Lzcm6.*m6.*t7-Lycm6.*Lz5.*m6.*t13-Lycm6.*Lzcm6.*m6.*t13);
et64 = t28.*(t79+t94+t97+t112+t113+t114+t166+t167+t177+t198+t235+t330+t333+t335+t343+t345+t347+t356+t357+t363+t375+t377+t387+t389+t425+t430+t457+t460+t474+t502+t503+t505+t514+t553+t556+t568+t570+t577+t580+t585+t589+t592+t596+t615+t619+t620+t628+t629+t630+t631+t641+t642+t660+t662+t665+t690+t692+t693+t694+t726+t732+t734+t742+t743+t760+t767+t768+t789+t793+t794+t797+t799+t814+t817+t850+t854+t855+t856+t857+t869+t883+t898+t900+t910+t914+t915+t917+t922+t924+t926+t934+t944+t945+t946+t947+t972+t973+t975+t978+t979+t980+t981+t983+t984+t988+t990+t992+t1001+t1009+t1025+t1036+t5.*t423-t5.*t470-Lx2.*t5.*t127-Lx2.*t5.*t128-Lx2.*t5.*t129+Lx2.*t5.*t136+Lx2.*Lxcm5.*m5.*t6.*t10+Lx2.*Lz5.*m6.*t10.*t12+Lx2.*Lzcm5.*m5.*t10.*t12+Lx2.*Lzcm6.*m6.*t10.*t12+Lx2.*Lxcm6.*m6.*t6.*t7.*t10-Lx2.*Lycm6.*m6.*t6.*t10.*t13);
et65 = t29.*(t79+t94+t97+t112+t113+t114+t166+t167+t177+t198+t235+t330+t333+t335+t343+t345+t347+t356+t357+t363+t375+t377+t387+t389+t425+t430+t457+t460+t474+t502+t503+t505+t514+t553+t556+t568+t570+t577+t580+t585+t589+t592+t596+t615+t619+t620+t628+t629+t630+t631+t641+t642+t660+t662+t665+t690+t692+t693+t694+t726+t732+t734+t742+t743+t760+t767+t768+t789+t793+t794+t797+t799+t814+t817+t850+t854+t855+t856+t857+t869+t883+t898+t900+t910+t914+t915+t917+t922+t924+t926+t934+t944+t945+t946+t947+t972+t973+t975+t978+t979+t980+t981+t983+t984+t988+t990+t992+t1001+t1009+t1025+t1036)-t30.*(t94+t97+t166+t167+t177+t330+t333+t335+t343+t345+t347+t356+t357+t363+t387+t389+t457+t460+t553+t556+t568+t570+t592+t596+t620+t628+t629+t630+t631+t690+t692+t693+t694+t768+t789+t917)+t27.*(et61+et62);
et66 = t31.*(t176+t329+t332-(Ixx6.*t39)./2.0+(Iyy6.*t39)./2.0+(m6.*t17.*t39)./2.0-(m6.*t20.*t39)./2.0)+t30.*(-t176-t329-t332+t371+t429+t432+t479+t481+t579+t582+t587+t591+t617+t703+t764+t807+t810+t888+t901+t902+t920+Ixx6.*t7.*t13-Iyy6.*t7.*t13-m6.*t7.*t13.*t17+m6.*t7.*t13.*t20);
et67 = -t27.*(t1078.*t1151.*(-1.0./2.0)-(t1078.*(Ixy6.*t1078+Iyy6.*(t321-t1043)))./2.0-(t1038.*(Ixz6.*t1078-Iyz6.*(t321-t1043)))./2.0+((t321-t1043).*(Ixx6.*t1078+Iyx6.*(t321-t1043)))./2.0+((t321-t1043).*(t1054-t1087+Ixy6.*(t321-t1043)))./2.0+m6.*t1183.*(Lycm6.*t1142-Lxcm6.*(t1075-t1128))+m6.*t1181.*(Lxcm6.*t1147+Lycm6.*(t1126-t13.*(t50-t1048))));
et68 = -t29.*(t242+t273+t281+t364+t371+t429+t432+t479+t481+t512+t579+t582+t587+t591+t617+t621+t677+t678+t696+t703+t709+t724+t744+t756+t764+t769+t784+t785+t804+t805+t807+t810+t812+t815+t848+t866+t867+t882+t886+t887+t888+t897+t899+t901+t902+t908+t913+t918+t920+t928+t955+t958+t976+t985+t986+t991+t993+t994+t995+t996+t998+t999+t1005+t1015+t1019+t1022+t1023+t1028+t1031+t1032+t1034);
et69 = -t28.*(t242+t273+t281+t364+t371+t429+t432+t479+t481+t512+t579+t582+t587+t591+t617+t621+t677+t678+t696+t703+t709+t724+t744+t756+t764+t769+t784+t785+t804+t805+t807+t810+t812+t815+t848+t866+t867+t882+t886+t887+t888+t897+t899+t901+t902+t908+t913+t918+t920+t928+t955+t958+t976+t985+t986+t991+t993+t994+t995+t996+t998+t999+t1005+t1015+t1019+t1022+t1023+t1028+t1031+t1032+t1034-Lx2.*Lxcm6.*m6.*t4.*t7.*t11+Lx2.*Lxcm6.*m6.*t10.*t12.*t13+Lx2.*Lycm6.*m6.*t4.*t11.*t13+Lx2.*Lycm6.*m6.*t7.*t10.*t12-Lx2.*Lxcm6.*m6.*t4.*t5.*t6.*t13-Lx2.*Lycm6.*m6.*t4.*t5.*t6.*t7);
out1 = [et1+et2+et3+et4+et5+et6+et7+et8+et9+et10+et11+et12+et13+et14+et15+et16+et17+et18+et19+et20+et21+et22+et23+et24+et25+et26+et27+et28+et29+et30+et31+et32+et33+et34+et35+et36+et37+et38+et39+et40+et41+et42+et43+et44+et45+et46+et47+et48+et49;et50+et51+et52;et53+et54;et58+et59+et60;et63+et64+et65;et66+et67+et68+et69];
end
